simulink model "model"  (R2016a)
(part 2 of 2)

  _CN_68186251_220000_CN_281815404_220000 : powerlib/Elements/Distributed Parameters Line  Phases=3  Frequency=50  Resistance=[0.01273 0.3864]  Inductance="[0.9337e-3  4.1264e-3]"  Capacitance=[12.74e-9 7.751e-9]  Length=9.6858  x1=[8.73114913702011e-11 380000 380000;314.159265358979 314.159265358979 314.159265358979;-0.177670123217348 0.415246442777429 -1.15554988401747]  x2=[1.26090477118469e-09 381852.398472139 381852.398472139;314.159265358979 314.159265358979 314.159265358979;-1.41941675517191 0.415007521738739 -1.15578880505616]  x3=[1.07663708898761e-11 1405.24743813465 1405.24743813466;314.159265358979 314.159265358979 314.159265358979;-2.70558821102223 0.316110507002444 -1.25468581979246]  x4=[8.62234243168895e-12 1405.96374414071 1405.9637441407;314.159265358979 314.159265358979 314.159265358979;0.245769282942371 0.405640215255436 -1.16515611153945]  x5=0.000565541566995742  V1=ones(3,3)  V2=ones(3,3)  I1=ones(3,3)  I2=ones(3,3)  nHarmo=1  Measurements=None
  _CN_68186251_220000_CN_376534298_220000 : powerlib/Elements/Distributed Parameters Line  Phases=3  Frequency=50  Resistance=[0.01273 0.3864]  Inductance="[0.9337e-3  4.1264e-3]"  Capacitance=[12.74e-9 7.751e-9]  Length=7.5155  x1=[8.73114913702011e-11 380000 380000;314.159265358979 314.159265358979 314.159265358979;-0.177670123217348 0.415246442777429 -1.15554988401747]  x2=[1.26090477118469e-09 381852.398472139 381852.398472139;314.159265358979 314.159265358979 314.159265358979;-1.41941675517191 0.415007521738739 -1.15578880505616]  x3=[1.07663708898761e-11 1405.24743813465 1405.24743813466;314.159265358979 314.159265358979 314.159265358979;-2.70558821102223 0.316110507002444 -1.25468581979246]  x4=[8.62234243168895e-12 1405.96374414071 1405.9637441407;314.159265358979 314.159265358979 314.159265358979;0.245769282942371 0.405640215255436 -1.16515611153945]  x5=0.000565541566995742  V1=ones(3,3)  V2=ones(3,3)  I1=ones(3,3)  I2=ones(3,3)  nHarmo=1  Measurements=None
  _CN_71500123_220000_CN_210568055_220000 : powerlib/Elements/Distributed Parameters Line  Phases=3  Frequency=50  Resistance=[0.01273 0.3864]  Inductance="[0.9337e-3  4.1264e-3]"  Capacitance=[12.74e-9 7.751e-9]  Length=40.5732  x1=[8.73114913702011e-11 380000 380000;314.159265358979 314.159265358979 314.159265358979;-0.177670123217348 0.415246442777429 -1.15554988401747]  x2=[1.26090477118469e-09 381852.398472139 381852.398472139;314.159265358979 314.159265358979 314.159265358979;-1.41941675517191 0.415007521738739 -1.15578880505616]  x3=[1.07663708898761e-11 1405.24743813465 1405.24743813466;314.159265358979 314.159265358979 314.159265358979;-2.70558821102223 0.316110507002444 -1.25468581979246]  x4=[8.62234243168895e-12 1405.96374414071 1405.9637441407;314.159265358979 314.159265358979 314.159265358979;0.245769282942371 0.405640215255436 -1.16515611153945]  x5=0.000565541566995742  V1=ones(3,3)  V2=ones(3,3)  I1=ones(3,3)  I2=ones(3,3)  nHarmo=1  Measurements=None
  _CN_71500123_220000_CN_211907009_220000 : powerlib/Elements/Distributed Parameters Line  Phases=3  Frequency=50  Resistance=[0.01273 0.3864]  Inductance="[0.9337e-3  4.1264e-3]"  Capacitance=[12.74e-9 7.751e-9]  Length=44.7884  x1=[8.73114913702011e-11 380000 380000;314.159265358979 314.159265358979 314.159265358979;-0.177670123217348 0.415246442777429 -1.15554988401747]  x2=[1.26090477118469e-09 381852.398472139 381852.398472139;314.159265358979 314.159265358979 314.159265358979;-1.41941675517191 0.415007521738739 -1.15578880505616]  x3=[1.07663708898761e-11 1405.24743813465 1405.24743813466;314.159265358979 314.159265358979 314.159265358979;-2.70558821102223 0.316110507002444 -1.25468581979246]  x4=[8.62234243168895e-12 1405.96374414071 1405.9637441407;314.159265358979 314.159265358979 314.159265358979;0.245769282942371 0.405640215255436 -1.16515611153945]  x5=0.000565541566995742  V1=ones(3,3)  V2=ones(3,3)  I1=ones(3,3)  I2=ones(3,3)  nHarmo=1  Measurements=None
  _CN_71500123_220000_CN_36348118_220000 : powerlib/Elements/Distributed Parameters Line  Phases=3  Frequency=50  Resistance=[0.01273 0.3864]  Inductance="[0.9337e-3  4.1264e-3]"  Capacitance=[12.74e-9 7.751e-9]  Length=9.2289  x1=[8.73114913702011e-11 380000 380000;314.159265358979 314.159265358979 314.159265358979;-0.177670123217348 0.415246442777429 -1.15554988401747]  x2=[1.26090477118469e-09 381852.398472139 381852.398472139;314.159265358979 314.159265358979 314.159265358979;-1.41941675517191 0.415007521738739 -1.15578880505616]  x3=[1.07663708898761e-11 1405.24743813465 1405.24743813466;314.159265358979 314.159265358979 314.159265358979;-2.70558821102223 0.316110507002444 -1.25468581979246]  x4=[8.62234243168895e-12 1405.96374414071 1405.9637441407;314.159265358979 314.159265358979 314.159265358979;0.245769282942371 0.405640215255436 -1.16515611153945]  x5=0.000565541566995742  V1=ones(3,3)  V2=ones(3,3)  I1=ones(3,3)  I2=ones(3,3)  nHarmo=1  Measurements=None
  _CN_71500123_220000_CN_365556107_220000 : powerlib/Elements/Distributed Parameters Line  Phases=3  Frequency=50  Resistance=[0.01273 0.3864]  Inductance="[0.9337e-3  4.1264e-3]"  Capacitance=[12.74e-9 7.751e-9]  Length=24.4165  x1=[8.73114913702011e-11 380000 380000;314.159265358979 314.159265358979 314.159265358979;-0.177670123217348 0.415246442777429 -1.15554988401747]  x2=[1.26090477118469e-09 381852.398472139 381852.398472139;314.159265358979 314.159265358979 314.159265358979;-1.41941675517191 0.415007521738739 -1.15578880505616]  x3=[1.07663708898761e-11 1405.24743813465 1405.24743813466;314.159265358979 314.159265358979 314.159265358979;-2.70558821102223 0.316110507002444 -1.25468581979246]  x4=[8.62234243168895e-12 1405.96374414071 1405.9637441407;314.159265358979 314.159265358979 314.159265358979;0.245769282942371 0.405640215255436 -1.16515611153945]  x5=0.000565541566995742  V1=ones(3,3)  V2=ones(3,3)  I1=ones(3,3)  I2=ones(3,3)  nHarmo=1  Measurements=None
  _CN_71500123_380000_CN156092814 : powerlib/Elements/Distributed Parameters Line  Phases=3  Frequency=50  Resistance=[0.01273 0.3864]  Inductance="[0.9337e-3  4.1264e-3]"  Capacitance=[12.74e-9 7.751e-9]  Length=26.701  x1=[8.73114913702011e-11 380000 380000;314.159265358979 314.159265358979 314.159265358979;-0.177670123217348 0.415246442777429 -1.15554988401747]  x2=[1.26090477118469e-09 381852.398472139 381852.398472139;314.159265358979 314.159265358979 314.159265358979;-1.41941675517191 0.415007521738739 -1.15578880505616]  x3=[1.07663708898761e-11 1405.24743813465 1405.24743813466;314.159265358979 314.159265358979 314.159265358979;-2.70558821102223 0.316110507002444 -1.25468581979246]  x4=[8.62234243168895e-12 1405.96374414071 1405.9637441407;314.159265358979 314.159265358979 314.159265358979;0.245769282942371 0.405640215255436 -1.16515611153945]  x5=0.000565541566995742  V1=ones(3,3)  V2=ones(3,3)  I1=ones(3,3)  I2=ones(3,3)  nHarmo=1  Measurements=None
  _CN_80266169_220000_CN_163881972_220000 : powerlib/Elements/Distributed Parameters Line  Phases=3  Frequency=50  Resistance=[0.01273 0.3864]  Inductance="[0.9337e-3  4.1264e-3]"  Capacitance=[12.74e-9 7.751e-9]  Length=17.0488  x1=[8.73114913702011e-11 380000 380000;314.159265358979 314.159265358979 314.159265358979;-0.177670123217348 0.415246442777429 -1.15554988401747]  x2=[1.26090477118469e-09 381852.398472139 381852.398472139;314.159265358979 314.159265358979 314.159265358979;-1.41941675517191 0.415007521738739 -1.15578880505616]  x3=[1.07663708898761e-11 1405.24743813465 1405.24743813466;314.159265358979 314.159265358979 314.159265358979;-2.70558821102223 0.316110507002444 -1.25468581979246]  x4=[8.62234243168895e-12 1405.96374414071 1405.9637441407;314.159265358979 314.159265358979 314.159265358979;0.245769282942371 0.405640215255436 -1.16515611153945]  x5=0.000565541566995742  V1=ones(3,3)  V2=ones(3,3)  I1=ones(3,3)  I2=ones(3,3)  nHarmo=1  Measurements=None
  _CN_80266169_220000_CN_194258388_220000 : powerlib/Elements/Distributed Parameters Line  Phases=3  Frequency=50  Resistance=[0.01273 0.3864]  Inductance="[0.9337e-3  4.1264e-3]"  Capacitance=[12.74e-9 7.751e-9]  Length=66.2326  x1=[8.73114913702011e-11 380000 380000;314.159265358979 314.159265358979 314.159265358979;-0.177670123217348 0.415246442777429 -1.15554988401747]  x2=[1.26090477118469e-09 381852.398472139 381852.398472139;314.159265358979 314.159265358979 314.159265358979;-1.41941675517191 0.415007521738739 -1.15578880505616]  x3=[1.07663708898761e-11 1405.24743813465 1405.24743813466;314.159265358979 314.159265358979 314.159265358979;-2.70558821102223 0.316110507002444 -1.25468581979246]  x4=[8.62234243168895e-12 1405.96374414071 1405.9637441407;314.159265358979 314.159265358979 314.159265358979;0.245769282942371 0.405640215255436 -1.16515611153945]  x5=0.000565541566995742  V1=ones(3,3)  V2=ones(3,3)  I1=ones(3,3)  I2=ones(3,3)  nHarmo=1  Measurements=None
  _CN_80266169_220000_CN_34238394_220000 : powerlib/Elements/Distributed Parameters Line  Phases=3  Frequency=50  Resistance=[0.01273 0.3864]  Inductance="[0.9337e-3  4.1264e-3]"  Capacitance=[12.74e-9 7.751e-9]  Length=1.2448  x1=[8.73114913702011e-11 380000 380000;314.159265358979 314.159265358979 314.159265358979;-0.177670123217348 0.415246442777429 -1.15554988401747]  x2=[1.26090477118469e-09 381852.398472139 381852.398472139;314.159265358979 314.159265358979 314.159265358979;-1.41941675517191 0.415007521738739 -1.15578880505616]  x3=[1.07663708898761e-11 1405.24743813465 1405.24743813466;314.159265358979 314.159265358979 314.159265358979;-2.70558821102223 0.316110507002444 -1.25468581979246]  x4=[8.62234243168895e-12 1405.96374414071 1405.9637441407;314.159265358979 314.159265358979 314.159265358979;0.245769282942371 0.405640215255436 -1.16515611153945]  x5=0.000565541566995742  V1=ones(3,3)  V2=ones(3,3)  I1=ones(3,3)  I2=ones(3,3)  nHarmo=1  Measurements=None
  _CN_89405664_220000_CN_190819048_220000 : powerlib/Elements/Distributed Parameters Line  Phases=3  Frequency=50  Resistance=[0.01273 0.3864]  Inductance="[0.9337e-3  4.1264e-3]"  Capacitance=[12.74e-9 7.751e-9]  Length=27.3541  x1=[8.73114913702011e-11 380000 380000;314.159265358979 314.159265358979 314.159265358979;-0.177670123217348 0.415246442777429 -1.15554988401747]  x2=[1.26090477118469e-09 381852.398472139 381852.398472139;314.159265358979 314.159265358979 314.159265358979;-1.41941675517191 0.415007521738739 -1.15578880505616]  x3=[1.07663708898761e-11 1405.24743813465 1405.24743813466;314.159265358979 314.159265358979 314.159265358979;-2.70558821102223 0.316110507002444 -1.25468581979246]  x4=[8.62234243168895e-12 1405.96374414071 1405.9637441407;314.159265358979 314.159265358979 314.159265358979;0.245769282942371 0.405640215255436 -1.16515611153945]  x5=0.000565541566995742  V1=ones(3,3)  V2=ones(3,3)  I1=ones(3,3)  I2=ones(3,3)  nHarmo=1  Measurements=None
  _CN_89977424_380000_CN_195751829_380000 : powerlib/Elements/Distributed Parameters Line  Phases=3  Frequency=50  Resistance=[0.01273 0.3864]  Inductance="[0.9337e-3  4.1264e-3]"  Capacitance=[12.74e-9 7.751e-9]  Length=3.0406  x1=[8.73114913702011e-11 380000 380000;314.159265358979 314.159265358979 314.159265358979;-0.177670123217348 0.415246442777429 -1.15554988401747]  x2=[1.26090477118469e-09 381852.398472139 381852.398472139;314.159265358979 314.159265358979 314.159265358979;-1.41941675517191 0.415007521738739 -1.15578880505616]  x3=[1.07663708898761e-11 1405.24743813465 1405.24743813466;314.159265358979 314.159265358979 314.159265358979;-2.70558821102223 0.316110507002444 -1.25468581979246]  x4=[8.62234243168895e-12 1405.96374414071 1405.9637441407;314.159265358979 314.159265358979 314.159265358979;0.245769282942371 0.405640215255436 -1.16515611153945]  x5=0.000565541566995742  V1=ones(3,3)  V2=ones(3,3)  I1=ones(3,3)  I2=ones(3,3)  nHarmo=1  Measurements=None
  _CN_89977424_380000_CN_31308888_380000 : powerlib/Elements/Distributed Parameters Line  Phases=3  Frequency=50  Resistance=[0.01273 0.3864]  Inductance="[0.9337e-3  4.1264e-3]"  Capacitance=[12.74e-9 7.751e-9]  Length=10.6473  x1=[8.73114913702011e-11 380000 380000;314.159265358979 314.159265358979 314.159265358979;-0.177670123217348 0.415246442777429 -1.15554988401747]  x2=[1.26090477118469e-09 381852.398472139 381852.398472139;314.159265358979 314.159265358979 314.159265358979;-1.41941675517191 0.415007521738739 -1.15578880505616]  x3=[1.07663708898761e-11 1405.24743813465 1405.24743813466;314.159265358979 314.159265358979 314.159265358979;-2.70558821102223 0.316110507002444 -1.25468581979246]  x4=[8.62234243168895e-12 1405.96374414071 1405.9637441407;314.159265358979 314.159265358979 314.159265358979;0.245769282942371 0.405640215255436 -1.16515611153945]  x5=0.000565541566995742  V1=ones(3,3)  V2=ones(3,3)  I1=ones(3,3)  I2=ones(3,3)  nHarmo=1  Measurements=None
  _CN_97941869_380000_CN_35002638_380000 : powerlib/Elements/Distributed Parameters Line  Phases=3  Frequency=50  Resistance=[0.01273 0.3864]  Inductance="[0.9337e-3  4.1264e-3]"  Capacitance=[12.74e-9 7.751e-9]  Length=18.8024  x1=[8.73114913702011e-11 380000 380000;314.159265358979 314.159265358979 314.159265358979;-0.177670123217348 0.415246442777429 -1.15554988401747]  x2=[1.26090477118469e-09 381852.398472139 381852.398472139;314.159265358979 314.159265358979 314.159265358979;-1.41941675517191 0.415007521738739 -1.15578880505616]  x3=[1.07663708898761e-11 1405.24743813465 1405.24743813466;314.159265358979 314.159265358979 314.159265358979;-2.70558821102223 0.316110507002444 -1.25468581979246]  x4=[8.62234243168895e-12 1405.96374414071 1405.9637441407;314.159265358979 314.159265358979 314.159265358979;0.245769282942371 0.405640215255436 -1.16515611153945]  x5=0.000565541566995742  V1=ones(3,3)  V2=ones(3,3)  I1=ones(3,3)  I2=ones(3,3)  nHarmo=1  Measurements=None
  _CN_98648381_220000_CN_27107779_220000 : powerlib/Elements/Distributed Parameters Line  Phases=3  Frequency=50  Resistance=[0.01273 0.3864]  Inductance="[0.9337e-3  4.1264e-3]"  Capacitance=[12.74e-9 7.751e-9]  Length=59.2829  x1=[8.73114913702011e-11 380000 380000;314.159265358979 314.159265358979 314.159265358979;-0.177670123217348 0.415246442777429 -1.15554988401747]  x2=[1.26090477118469e-09 381852.398472139 381852.398472139;314.159265358979 314.159265358979 314.159265358979;-1.41941675517191 0.415007521738739 -1.15578880505616]  x3=[1.07663708898761e-11 1405.24743813465 1405.24743813466;314.159265358979 314.159265358979 314.159265358979;-2.70558821102223 0.316110507002444 -1.25468581979246]  x4=[8.62234243168895e-12 1405.96374414071 1405.9637441407;314.159265358979 314.159265358979 314.159265358979;0.245769282942371 0.405640215255436 -1.16515611153945]  x5=0.000565541566995742  V1=ones(3,3)  V2=ones(3,3)  I1=ones(3,3)  I2=ones(3,3)  nHarmo=1  Measurements=None
  _CN_98648381_220000_CN_50319857_220000 : powerlib/Elements/Distributed Parameters Line  Phases=3  Frequency=50  Resistance=[0.01273 0.3864]  Inductance="[0.9337e-3  4.1264e-3]"  Capacitance=[12.74e-9 7.751e-9]  Length=22.8534  x1=[8.73114913702011e-11 380000 380000;314.159265358979 314.159265358979 314.159265358979;-0.177670123217348 0.415246442777429 -1.15554988401747]  x2=[1.26090477118469e-09 381852.398472139 381852.398472139;314.159265358979 314.159265358979 314.159265358979;-1.41941675517191 0.415007521738739 -1.15578880505616]  x3=[1.07663708898761e-11 1405.24743813465 1405.24743813466;314.159265358979 314.159265358979 314.159265358979;-2.70558821102223 0.316110507002444 -1.25468581979246]  x4=[8.62234243168895e-12 1405.96374414071 1405.9637441407;314.159265358979 314.159265358979 314.159265358979;0.245769282942371 0.405640215255436 -1.16515611153945]  x5=0.000565541566995742  V1=ones(3,3)  V2=ones(3,3)  I1=ones(3,3)  I2=ones(3,3)  nHarmo=1  Measurements=None
  _CN_98648381_380000_CN_147714395_380000 : powerlib/Elements/Distributed Parameters Line  Phases=3  Frequency=50  Resistance=[0.01273 0.3864]  Inductance="[0.9337e-3  4.1264e-3]"  Capacitance=[12.74e-9 7.751e-9]  Length=59.2296  x1=[8.73114913702011e-11 380000 380000;314.159265358979 314.159265358979 314.159265358979;-0.177670123217348 0.415246442777429 -1.15554988401747]  x2=[1.26090477118469e-09 381852.398472139 381852.398472139;314.159265358979 314.159265358979 314.159265358979;-1.41941675517191 0.415007521738739 -1.15578880505616]  x3=[1.07663708898761e-11 1405.24743813465 1405.24743813466;314.159265358979 314.159265358979 314.159265358979;-2.70558821102223 0.316110507002444 -1.25468581979246]  x4=[8.62234243168895e-12 1405.96374414071 1405.9637441407;314.159265358979 314.159265358979 314.159265358979;0.245769282942371 0.405640215255436 -1.16515611153945]  x5=0.000565541566995742  V1=ones(3,3)  V2=ones(3,3)  I1=ones(3,3)  I2=ones(3,3)  nHarmo=1  Measurements=None
  _CN_98648381_380000_CN_50319857_380000 : powerlib/Elements/Distributed Parameters Line  Phases=3  Frequency=50  Resistance=[0.01273 0.3864]  Inductance="[0.9337e-3  4.1264e-3]"  Capacitance=[12.74e-9 7.751e-9]  Length=22.6956  x1=[8.73114913702011e-11 380000 380000;314.159265358979 314.159265358979 314.159265358979;-0.177670123217348 0.415246442777429 -1.15554988401747]  x2=[1.26090477118469e-09 381852.398472139 381852.398472139;314.159265358979 314.159265358979 314.159265358979;-1.41941675517191 0.415007521738739 -1.15578880505616]  x3=[1.07663708898761e-11 1405.24743813465 1405.24743813466;314.159265358979 314.159265358979 314.159265358979;-2.70558821102223 0.316110507002444 -1.25468581979246]  x4=[8.62234243168895e-12 1405.96374414071 1405.9637441407;314.159265358979 314.159265358979 314.159265358979;0.245769282942371 0.405640215255436 -1.16515611153945]  x5=0.000565541566995742  V1=ones(3,3)  V2=ones(3,3)  I1=ones(3,3)  I2=ones(3,3)  nHarmo=1  Measurements=None
  bus1 : powerlib/Measurements/Load Flow Bus  LConnTagsString=a  Phases=single  Connectors=on one side  ID=bus1  Vbase=220000  Vref=1  Vangle=0  VLF=1  VLFb=1  VLFc=1  angleLF=0  angleLFb=0  angleLFc=0
      settings: AttributesFormatString=|
      | %<ID>
      | %<Vbase>V
      | %<VLF>pu
      | %<angleLF>deg.
      | %<Name>
  bus10 : powerlib/Measurements/Load Flow Bus  LConnTagsString=a  Phases=single  Connectors=on one side  ID=bus10  Vbase=220000  Vref=1  Vangle=0  VLF=1  VLFb=1  VLFc=1  angleLF=0  angleLFb=0  angleLFc=0
      settings: AttributesFormatString=|
      | %<ID>
      | %<Vbase>V
      | %<VLF>pu
      | %<angleLF>deg.
      | %<Name>
  bus100 : powerlib/Measurements/Load Flow Bus  LConnTagsString=a  Phases=single  Connectors=on one side  ID=bus100  Vbase=220000  Vref=1  Vangle=0  VLF=1  VLFb=1  VLFc=1  angleLF=0  angleLFb=0  angleLFc=0
      settings: AttributesFormatString=|
      | %<ID>
      | %<Vbase>V
      | %<VLF>pu
      | %<angleLF>deg.
      | %<Name>
  bus101 : powerlib/Measurements/Load Flow Bus  LConnTagsString=a  Phases=single  Connectors=on one side  ID=bus101  Vbase=220000  Vref=1  Vangle=0  VLF=1  VLFb=1  VLFc=1  angleLF=0  angleLFb=0  angleLFc=0
      settings: AttributesFormatString=|
      | %<ID>
      | %<Vbase>V
      | %<VLF>pu
      | %<angleLF>deg.
      | %<Name>
  bus102 : powerlib/Measurements/Load Flow Bus  LConnTagsString=a  Phases=single  Connectors=on one side  ID=bus102  Vbase=220000  Vref=1  Vangle=0  VLF=1  VLFb=1  VLFc=1  angleLF=0  angleLFb=0  angleLFc=0
      settings: AttributesFormatString=|
      | %<ID>
      | %<Vbase>V
      | %<VLF>pu
      | %<angleLF>deg.
      | %<Name>
  bus103 : powerlib/Measurements/Load Flow Bus  LConnTagsString=a  Phases=single  Connectors=on one side  ID=bus103  Vbase=220000  Vref=1  Vangle=0  VLF=1  VLFb=1  VLFc=1  angleLF=0  angleLFb=0  angleLFc=0
      settings: AttributesFormatString=|
      | %<ID>
      | %<Vbase>V
      | %<VLF>pu
      | %<angleLF>deg.
      | %<Name>
  bus104 : powerlib/Measurements/Load Flow Bus  LConnTagsString=a  Phases=single  Connectors=on one side  ID=bus104  Vbase=220000  Vref=1  Vangle=0  VLF=1  VLFb=1  VLFc=1  angleLF=0  angleLFb=0  angleLFc=0
      settings: AttributesFormatString=|
      | %<ID>
      | %<Vbase>V
      | %<VLF>pu
      | %<angleLF>deg.
      | %<Name>
  bus105 : powerlib/Measurements/Load Flow Bus  LConnTagsString=a  Phases=single  Connectors=on one side  ID=bus105  Vbase=220000  Vref=1  Vangle=0  VLF=1  VLFb=1  VLFc=1  angleLF=0  angleLFb=0  angleLFc=0
      settings: AttributesFormatString=|
      | %<ID>
      | %<Vbase>V
      | %<VLF>pu
      | %<angleLF>deg.
      | %<Name>
  bus106 : powerlib/Measurements/Load Flow Bus  LConnTagsString=a  Phases=single  Connectors=on one side  ID=bus106  Vbase=380000  Vref=1  Vangle=0  VLF=1  VLFb=1  VLFc=1  angleLF=0  angleLFb=0  angleLFc=0
      settings: AttributesFormatString=|
      | %<ID>
      | %<Vbase>V
      | %<VLF>pu
      | %<angleLF>deg.
      | %<Name>
  bus107 : powerlib/Measurements/Load Flow Bus  LConnTagsString=a  Phases=single  Connectors=on one side  ID=bus107  Vbase=220000  Vref=1  Vangle=0  VLF=1  VLFb=1  VLFc=1  angleLF=0  angleLFb=0  angleLFc=0
      settings: AttributesFormatString=|
      | %<ID>
      | %<Vbase>V
      | %<VLF>pu
      | %<angleLF>deg.
      | %<Name>
  bus108 : powerlib/Measurements/Load Flow Bus  LConnTagsString=a  Phases=single  Connectors=on one side  ID=bus108  Vbase=220000  Vref=1  Vangle=0  VLF=1  VLFb=1  VLFc=1  angleLF=0  angleLFb=0  angleLFc=0
      settings: AttributesFormatString=|
      | %<ID>
      | %<Vbase>V
      | %<VLF>pu
      | %<angleLF>deg.
      | %<Name>
  bus109 : powerlib/Measurements/Load Flow Bus  LConnTagsString=a  Phases=single  Connectors=on one side  ID=bus109  Vbase=220000  Vref=1  Vangle=0  VLF=1  VLFb=1  VLFc=1  angleLF=0  angleLFb=0  angleLFc=0
      settings: AttributesFormatString=|
      | %<ID>
      | %<Vbase>V
      | %<VLF>pu
      | %<angleLF>deg.
      | %<Name>
  bus11 : powerlib/Measurements/Load Flow Bus  LConnTagsString=a  Phases=single  Connectors=on one side  ID=bus11  Vbase=220000  Vref=1  Vangle=0  VLF=1  VLFb=1  VLFc=1  angleLF=0  angleLFb=0  angleLFc=0
      settings: AttributesFormatString=|
      | %<ID>
      | %<Vbase>V
      | %<VLF>pu
      | %<angleLF>deg.
      | %<Name>
  bus110 : powerlib/Measurements/Load Flow Bus  LConnTagsString=a  Phases=single  Connectors=on one side  ID=bus110  Vbase=220000  Vref=1  Vangle=0  VLF=1  VLFb=1  VLFc=1  angleLF=0  angleLFb=0  angleLFc=0
      settings: AttributesFormatString=|
      | %<ID>
      | %<Vbase>V
      | %<VLF>pu
      | %<angleLF>deg.
      | %<Name>
  bus111 : powerlib/Measurements/Load Flow Bus  LConnTagsString=a  Phases=single  Connectors=on one side  ID=bus111  Vbase=380000  Vref=1  Vangle=0  VLF=1  VLFb=1  VLFc=1  angleLF=0  angleLFb=0  angleLFc=0
      settings: AttributesFormatString=|
      | %<ID>
      | %<Vbase>V
      | %<VLF>pu
      | %<angleLF>deg.
      | %<Name>
  bus112 : powerlib/Measurements/Load Flow Bus  LConnTagsString=a  Phases=single  Connectors=on one side  ID=bus112  Vbase=380000  Vref=1  Vangle=0  VLF=1  VLFb=1  VLFc=1  angleLF=0  angleLFb=0  angleLFc=0
      settings: AttributesFormatString=|
      | %<ID>
      | %<Vbase>V
      | %<VLF>pu
      | %<angleLF>deg.
      | %<Name>
  bus113 : powerlib/Measurements/Load Flow Bus  LConnTagsString=a  Phases=single  Connectors=on one side  ID=bus113  Vbase=220000  Vref=1  Vangle=0  VLF=1  VLFb=1  VLFc=1  angleLF=0  angleLFb=0  angleLFc=0
      settings: AttributesFormatString=|
      | %<ID>
      | %<Vbase>V
      | %<VLF>pu
      | %<angleLF>deg.
      | %<Name>
  bus114 : powerlib/Measurements/Load Flow Bus  LConnTagsString=a  Phases=single  Connectors=on one side  ID=bus114  Vbase=220000  Vref=1  Vangle=0  VLF=1  VLFb=1  VLFc=1  angleLF=0  angleLFb=0  angleLFc=0
      settings: AttributesFormatString=|
      | %<ID>
      | %<Vbase>V
      | %<VLF>pu
      | %<angleLF>deg.
      | %<Name>
  bus115 : powerlib/Measurements/Load Flow Bus  LConnTagsString=a  Phases=single  Connectors=on one side  ID=bus115  Vbase=220000  Vref=1  Vangle=0  VLF=1  VLFb=1  VLFc=1  angleLF=0  angleLFb=0  angleLFc=0
      settings: AttributesFormatString=|
      | %<ID>
      | %<Vbase>V
      | %<VLF>pu
      | %<angleLF>deg.
      | %<Name>
  bus116 : powerlib/Measurements/Load Flow Bus  LConnTagsString=a  Phases=single  Connectors=on one side  ID=bus116  Vbase=220000  Vref=1  Vangle=0  VLF=1  VLFb=1  VLFc=1  angleLF=0  angleLFb=0  angleLFc=0
      settings: AttributesFormatString=|
      | %<ID>
      | %<Vbase>V
      | %<VLF>pu
      | %<angleLF>deg.
      | %<Name>
  bus117 : powerlib/Measurements/Load Flow Bus  LConnTagsString=a  Phases=single  Connectors=on one side  ID=bus117  Vbase=220000  Vref=1  Vangle=0  VLF=1  VLFb=1  VLFc=1  angleLF=0  angleLFb=0  angleLFc=0
      settings: AttributesFormatString=|
      | %<ID>
      | %<Vbase>V
      | %<VLF>pu
      | %<angleLF>deg.
      | %<Name>
  bus118 : powerlib/Measurements/Load Flow Bus  LConnTagsString=a  Phases=single  Connectors=on one side  ID=bus118  Vbase=220000  Vref=1  Vangle=0  VLF=1  VLFb=1  VLFc=1  angleLF=0  angleLFb=0  angleLFc=0
      settings: AttributesFormatString=|
      | %<ID>
      | %<Vbase>V
      | %<VLF>pu
      | %<angleLF>deg.
      | %<Name>
  bus119 : powerlib/Measurements/Load Flow Bus  LConnTagsString=a  Phases=single  Connectors=on one side  ID=bus119  Vbase=220000  Vref=1  Vangle=0  VLF=1  VLFb=1  VLFc=1  angleLF=0  angleLFb=0  angleLFc=0
      settings: AttributesFormatString=|
      | %<ID>
      | %<Vbase>V
      | %<VLF>pu
      | %<angleLF>deg.
      | %<Name>
  bus12 : powerlib/Measurements/Load Flow Bus  LConnTagsString=a  Phases=single  Connectors=on one side  ID=bus12  Vbase=220000  Vref=1  Vangle=0  VLF=1  VLFb=1  VLFc=1  angleLF=0  angleLFb=0  angleLFc=0
      settings: AttributesFormatString=|
      | %<ID>
      | %<Vbase>V
      | %<VLF>pu
      | %<angleLF>deg.
      | %<Name>
  bus120 : powerlib/Measurements/Load Flow Bus  LConnTagsString=a  Phases=single  Connectors=on one side  ID=bus120  Vbase=220000  Vref=1  Vangle=0  VLF=1  VLFb=1  VLFc=1  angleLF=0  angleLFb=0  angleLFc=0
      settings: AttributesFormatString=|
      | %<ID>
      | %<Vbase>V
      | %<VLF>pu
      | %<angleLF>deg.
      | %<Name>
  bus121 : powerlib/Measurements/Load Flow Bus  LConnTagsString=a  Phases=single  Connectors=on one side  ID=bus121  Vbase=220000  Vref=1  Vangle=0  VLF=1  VLFb=1  VLFc=1  angleLF=0  angleLFb=0  angleLFc=0
      settings: AttributesFormatString=|
      | %<ID>
      | %<Vbase>V
      | %<VLF>pu
      | %<angleLF>deg.
      | %<Name>
  bus122 : powerlib/Measurements/Load Flow Bus  LConnTagsString=a  Phases=single  Connectors=on one side  ID=bus122  Vbase=220000  Vref=1  Vangle=0  VLF=1  VLFb=1  VLFc=1  angleLF=0  angleLFb=0  angleLFc=0
      settings: AttributesFormatString=|
      | %<ID>
      | %<Vbase>V
      | %<VLF>pu
      | %<angleLF>deg.
      | %<Name>
  bus123 : powerlib/Measurements/Load Flow Bus  LConnTagsString=a  Phases=single  Connectors=on one side  ID=bus123  Vbase=220000  Vref=1  Vangle=0  VLF=1  VLFb=1  VLFc=1  angleLF=0  angleLFb=0  angleLFc=0
      settings: AttributesFormatString=|
      | %<ID>
      | %<Vbase>V
      | %<VLF>pu
      | %<angleLF>deg.
      | %<Name>
  bus124 : powerlib/Measurements/Load Flow Bus  LConnTagsString=a  Phases=single  Connectors=on one side  ID=bus124  Vbase=220000  Vref=1  Vangle=0  VLF=1  VLFb=1  VLFc=1  angleLF=0  angleLFb=0  angleLFc=0
      settings: AttributesFormatString=|
      | %<ID>
      | %<Vbase>V
      | %<VLF>pu
      | %<angleLF>deg.
      | %<Name>
  bus125 : powerlib/Measurements/Load Flow Bus  LConnTagsString=a  Phases=single  Connectors=on one side  ID=bus125  Vbase=220000  Vref=1  Vangle=0  VLF=1  VLFb=1  VLFc=1  angleLF=0  angleLFb=0  angleLFc=0
      settings: AttributesFormatString=|
      | %<ID>
      | %<Vbase>V
      | %<VLF>pu
      | %<angleLF>deg.
      | %<Name>
  bus126 : powerlib/Measurements/Load Flow Bus  LConnTagsString=a  Phases=single  Connectors=on one side  ID=bus126  Vbase=220000  Vref=1  Vangle=0  VLF=1  VLFb=1  VLFc=1  angleLF=0  angleLFb=0  angleLFc=0
      settings: AttributesFormatString=|
      | %<ID>
      | %<Vbase>V
      | %<VLF>pu
      | %<angleLF>deg.
      | %<Name>
  bus127 : powerlib/Measurements/Load Flow Bus  LConnTagsString=a  Phases=single  Connectors=on one side  ID=bus127  Vbase=220000  Vref=1  Vangle=0  VLF=1  VLFb=1  VLFc=1  angleLF=0  angleLFb=0  angleLFc=0
      settings: AttributesFormatString=|
      | %<ID>
      | %<Vbase>V
      | %<VLF>pu
      | %<angleLF>deg.
      | %<Name>
  bus128 : powerlib/Measurements/Load Flow Bus  LConnTagsString=a  Phases=single  Connectors=on one side  ID=bus128  Vbase=220000  Vref=1  Vangle=0  VLF=1  VLFb=1  VLFc=1  angleLF=0  angleLFb=0  angleLFc=0
      settings: AttributesFormatString=|
      | %<ID>
      | %<Vbase>V
      | %<VLF>pu
      | %<angleLF>deg.
      | %<Name>
  bus129 : powerlib/Measurements/Load Flow Bus  LConnTagsString=a  Phases=single  Connectors=on one side  ID=bus129  Vbase=220000  Vref=1  Vangle=0  VLF=1  VLFb=1  VLFc=1  angleLF=0  angleLFb=0  angleLFc=0
      settings: AttributesFormatString=|
      | %<ID>
      | %<Vbase>V
      | %<VLF>pu
      | %<angleLF>deg.
      | %<Name>
  bus13 : powerlib/Measurements/Load Flow Bus  LConnTagsString=a  Phases=single  Connectors=on one side  ID=bus13  Vbase=220000  Vref=1  Vangle=0  VLF=1  VLFb=1  VLFc=1  angleLF=0  angleLFb=0  angleLFc=0
      settings: AttributesFormatString=|
      | %<ID>
      | %<Vbase>V
      | %<VLF>pu
      | %<angleLF>deg.
      | %<Name>
  bus130 : powerlib/Measurements/Load Flow Bus  LConnTagsString=a  Phases=single  Connectors=on one side  ID=bus130  Vbase=220000  Vref=1  Vangle=0  VLF=1  VLFb=1  VLFc=1  angleLF=0  angleLFb=0  angleLFc=0
      settings: AttributesFormatString=|
      | %<ID>
      | %<Vbase>V
      | %<VLF>pu
      | %<angleLF>deg.
      | %<Name>
  bus131 : powerlib/Measurements/Load Flow Bus  LConnTagsString=a  Phases=single  Connectors=on one side  ID=bus131  Vbase=220000  Vref=1  Vangle=0  VLF=1  VLFb=1  VLFc=1  angleLF=0  angleLFb=0  angleLFc=0
      settings: AttributesFormatString=|
      | %<ID>
      | %<Vbase>V
      | %<VLF>pu
      | %<angleLF>deg.
      | %<Name>
  bus132 : powerlib/Measurements/Load Flow Bus  LConnTagsString=a  Phases=single  Connectors=on one side  ID=bus132  Vbase=220000  Vref=1  Vangle=0  VLF=1  VLFb=1  VLFc=1  angleLF=0  angleLFb=0  angleLFc=0
      settings: AttributesFormatString=|
      | %<ID>
      | %<Vbase>V
      | %<VLF>pu
      | %<angleLF>deg.
      | %<Name>
  bus133 : powerlib/Measurements/Load Flow Bus  LConnTagsString=a  Phases=single  Connectors=on one side  ID=bus133  Vbase=220000  Vref=1  Vangle=0  VLF=1  VLFb=1  VLFc=1  angleLF=0  angleLFb=0  angleLFc=0
      settings: AttributesFormatString=|
      | %<ID>
      | %<Vbase>V
      | %<VLF>pu
      | %<angleLF>deg.
      | %<Name>
  bus134 : powerlib/Measurements/Load Flow Bus  LConnTagsString=a  Phases=single  Connectors=on one side  ID=bus134  Vbase=380000  Vref=1  Vangle=0  VLF=1  VLFb=1  VLFc=1  angleLF=0  angleLFb=0  angleLFc=0
      settings: AttributesFormatString=|
      | %<ID>
      | %<Vbase>V
      | %<VLF>pu
      | %<angleLF>deg.
      | %<Name>
  bus135 : powerlib/Measurements/Load Flow Bus  LConnTagsString=a  Phases=single  Connectors=on one side  ID=bus135  Vbase=380000  Vref=1  Vangle=0  VLF=1  VLFb=1  VLFc=1  angleLF=0  angleLFb=0  angleLFc=0
      settings: AttributesFormatString=|
      | %<ID>
      | %<Vbase>V
      | %<VLF>pu
      | %<angleLF>deg.
      | %<Name>
  bus136 : powerlib/Measurements/Load Flow Bus  LConnTagsString=a  Phases=single  Connectors=on one side  ID=bus136  Vbase=380000  Vref=1  Vangle=0  VLF=1  VLFb=1  VLFc=1  angleLF=0  angleLFb=0  angleLFc=0
      settings: AttributesFormatString=|
      | %<ID>
      | %<Vbase>V
      | %<VLF>pu
      | %<angleLF>deg.
      | %<Name>
  bus137 : powerlib/Measurements/Load Flow Bus  LConnTagsString=a  Phases=single  Connectors=on one side  ID=bus137  Vbase=220000  Vref=1  Vangle=0  VLF=1  VLFb=1  VLFc=1  angleLF=0  angleLFb=0  angleLFc=0
      settings: AttributesFormatString=|
      | %<ID>
      | %<Vbase>V
      | %<VLF>pu
      | %<angleLF>deg.
      | %<Name>
  bus138 : powerlib/Measurements/Load Flow Bus  LConnTagsString=a  Phases=single  Connectors=on one side  ID=bus138  Vbase=220000  Vref=1  Vangle=0  VLF=1  VLFb=1  VLFc=1  angleLF=0  angleLFb=0  angleLFc=0
      settings: AttributesFormatString=|
      | %<ID>
      | %<Vbase>V
      | %<VLF>pu
      | %<angleLF>deg.
      | %<Name>
  bus139 : powerlib/Measurements/Load Flow Bus  LConnTagsString=a  Phases=single  Connectors=on one side  ID=bus139  Vbase=220000  Vref=1  Vangle=0  VLF=1  VLFb=1  VLFc=1  angleLF=0  angleLFb=0  angleLFc=0
      settings: AttributesFormatString=|
      | %<ID>
      | %<Vbase>V
      | %<VLF>pu
      | %<angleLF>deg.
      | %<Name>
  bus14 : powerlib/Measurements/Load Flow Bus  LConnTagsString=a  Phases=single  Connectors=on one side  ID=bus14  Vbase=220000  Vref=1  Vangle=0  VLF=1  VLFb=1  VLFc=1  angleLF=0  angleLFb=0  angleLFc=0
      settings: AttributesFormatString=|
      | %<ID>
      | %<Vbase>V
      | %<VLF>pu
      | %<angleLF>deg.
      | %<Name>
  bus140 : powerlib/Measurements/Load Flow Bus  LConnTagsString=a  Phases=single  Connectors=on one side  ID=bus140  Vbase=220000  Vref=1  Vangle=0  VLF=1  VLFb=1  VLFc=1  angleLF=0  angleLFb=0  angleLFc=0
      settings: AttributesFormatString=|
      | %<ID>
      | %<Vbase>V
      | %<VLF>pu
      | %<angleLF>deg.
      | %<Name>
  bus141 : powerlib/Measurements/Load Flow Bus  LConnTagsString=a  Phases=single  Connectors=on one side  ID=bus141  Vbase=220000  Vref=1  Vangle=0  VLF=1  VLFb=1  VLFc=1  angleLF=0  angleLFb=0  angleLFc=0
      settings: AttributesFormatString=|
      | %<ID>
      | %<Vbase>V
      | %<VLF>pu
      | %<angleLF>deg.
      | %<Name>
  bus142 : powerlib/Measurements/Load Flow Bus  LConnTagsString=a  Phases=single  Connectors=on one side  ID=bus142  Vbase=220000  Vref=1  Vangle=0  VLF=1  VLFb=1  VLFc=1  angleLF=0  angleLFb=0  angleLFc=0
      settings: AttributesFormatString=|
      | %<ID>
      | %<Vbase>V
      | %<VLF>pu
      | %<angleLF>deg.
      | %<Name>
  bus143 : powerlib/Measurements/Load Flow Bus  LConnTagsString=a  Phases=single  Connectors=on one side  ID=bus143  Vbase=220000  Vref=1  Vangle=0  VLF=1  VLFb=1  VLFc=1  angleLF=0  angleLFb=0  angleLFc=0
      settings: AttributesFormatString=|
      | %<ID>
      | %<Vbase>V
      | %<VLF>pu
      | %<angleLF>deg.
      | %<Name>
  bus144 : powerlib/Measurements/Load Flow Bus  LConnTagsString=a  Phases=single  Connectors=on one side  ID=bus144  Vbase=220000  Vref=1  Vangle=0  VLF=1  VLFb=1  VLFc=1  angleLF=0  angleLFb=0  angleLFc=0
      settings: AttributesFormatString=|
      | %<ID>
      | %<Vbase>V
      | %<VLF>pu
      | %<angleLF>deg.
      | %<Name>
  bus145 : powerlib/Measurements/Load Flow Bus  LConnTagsString=a  Phases=single  Connectors=on one side  ID=bus145  Vbase=220000  Vref=1  Vangle=0  VLF=1  VLFb=1  VLFc=1  angleLF=0  angleLFb=0  angleLFc=0
      settings: AttributesFormatString=|
      | %<ID>
      | %<Vbase>V
      | %<VLF>pu
      | %<angleLF>deg.
      | %<Name>
  bus146 : powerlib/Measurements/Load Flow Bus  LConnTagsString=a  Phases=single  Connectors=on one side  ID=bus146  Vbase=220000  Vref=1  Vangle=0  VLF=1  VLFb=1  VLFc=1  angleLF=0  angleLFb=0  angleLFc=0
      settings: AttributesFormatString=|
      | %<ID>
      | %<Vbase>V
      | %<VLF>pu
      | %<angleLF>deg.
      | %<Name>
  bus147 : powerlib/Measurements/Load Flow Bus  LConnTagsString=a  Phases=single  Connectors=on one side  ID=bus147  Vbase=220000  Vref=1  Vangle=0  VLF=1  VLFb=1  VLFc=1  angleLF=0  angleLFb=0  angleLFc=0
      settings: AttributesFormatString=|
      | %<ID>
      | %<Vbase>V
      | %<VLF>pu
      | %<angleLF>deg.
      | %<Name>
  bus148 : powerlib/Measurements/Load Flow Bus  LConnTagsString=a  Phases=single  Connectors=on one side  ID=bus148  Vbase=380000  Vref=1  Vangle=0  VLF=1  VLFb=1  VLFc=1  angleLF=0  angleLFb=0  angleLFc=0
      settings: AttributesFormatString=|
      | %<ID>
      | %<Vbase>V
      | %<VLF>pu
      | %<angleLF>deg.
      | %<Name>
  bus149 : powerlib/Measurements/Load Flow Bus  LConnTagsString=a  Phases=single  Connectors=on one side  ID=bus149  Vbase=220000  Vref=1  Vangle=0  VLF=1  VLFb=1  VLFc=1  angleLF=0  angleLFb=0  angleLFc=0
      settings: AttributesFormatString=|
      | %<ID>
      | %<Vbase>V
      | %<VLF>pu
      | %<angleLF>deg.
      | %<Name>
  bus15 : powerlib/Measurements/Load Flow Bus  LConnTagsString=a  Phases=single  Connectors=on one side  ID=bus15  Vbase=220000  Vref=1  Vangle=0  VLF=1  VLFb=1  VLFc=1  angleLF=0  angleLFb=0  angleLFc=0
      settings: AttributesFormatString=|
      | %<ID>
      | %<Vbase>V
      | %<VLF>pu
      | %<angleLF>deg.
      | %<Name>
  bus150 : powerlib/Measurements/Load Flow Bus  LConnTagsString=a  Phases=single  Connectors=on one side  ID=bus150  Vbase=220000  Vref=1  Vangle=0  VLF=1  VLFb=1  VLFc=1  angleLF=0  angleLFb=0  angleLFc=0
      settings: AttributesFormatString=|
      | %<ID>
      | %<Vbase>V
      | %<VLF>pu
      | %<angleLF>deg.
      | %<Name>
  bus151 : powerlib/Measurements/Load Flow Bus  LConnTagsString=a  Phases=single  Connectors=on one side  ID=bus151  Vbase=220000  Vref=1  Vangle=0  VLF=1  VLFb=1  VLFc=1  angleLF=0  angleLFb=0  angleLFc=0
      settings: AttributesFormatString=|
      | %<ID>
      | %<Vbase>V
      | %<VLF>pu
      | %<angleLF>deg.
      | %<Name>
  bus152 : powerlib/Measurements/Load Flow Bus  LConnTagsString=a  Phases=single  Connectors=on one side  ID=bus152  Vbase=220000  Vref=1  Vangle=0  VLF=1  VLFb=1  VLFc=1  angleLF=0  angleLFb=0  angleLFc=0
      settings: AttributesFormatString=|
      | %<ID>
      | %<Vbase>V
      | %<VLF>pu
      | %<angleLF>deg.
      | %<Name>
  bus153 : powerlib/Measurements/Load Flow Bus  LConnTagsString=a  Phases=single  Connectors=on one side  ID=bus153  Vbase=380000  Vref=1  Vangle=0  VLF=1  VLFb=1  VLFc=1  angleLF=0  angleLFb=0  angleLFc=0
      settings: AttributesFormatString=|
      | %<ID>
      | %<Vbase>V
      | %<VLF>pu
      | %<angleLF>deg.
      | %<Name>
  bus154 : powerlib/Measurements/Load Flow Bus  LConnTagsString=a  Phases=single  Connectors=on one side  ID=bus154  Vbase=380000  Vref=1  Vangle=0  VLF=1  VLFb=1  VLFc=1  angleLF=0  angleLFb=0  angleLFc=0
      settings: AttributesFormatString=|
      | %<ID>
      | %<Vbase>V
      | %<VLF>pu
      | %<angleLF>deg.
      | %<Name>
  bus155 : powerlib/Measurements/Load Flow Bus  LConnTagsString=a  Phases=single  Connectors=on one side  ID=bus155  Vbase=380000  Vref=1  Vangle=0  VLF=1  VLFb=1  VLFc=1  angleLF=0  angleLFb=0  angleLFc=0
      settings: AttributesFormatString=|
      | %<ID>
      | %<Vbase>V
      | %<VLF>pu
      | %<angleLF>deg.
      | %<Name>
  bus156 : powerlib/Measurements/Load Flow Bus  LConnTagsString=a  Phases=single  Connectors=on one side  ID=bus156  Vbase=220000  Vref=1  Vangle=0  VLF=1  VLFb=1  VLFc=1  angleLF=0  angleLFb=0  angleLFc=0
      settings: AttributesFormatString=|
      | %<ID>
      | %<Vbase>V
      | %<VLF>pu
      | %<angleLF>deg.
      | %<Name>
  bus157 : powerlib/Measurements/Load Flow Bus  LConnTagsString=a  Phases=single  Connectors=on one side  ID=bus157  Vbase=220000  Vref=1  Vangle=0  VLF=1  VLFb=1  VLFc=1  angleLF=0  angleLFb=0  angleLFc=0
      settings: AttributesFormatString=|
      | %<ID>
      | %<Vbase>V
      | %<VLF>pu
      | %<angleLF>deg.
      | %<Name>
  bus158 : powerlib/Measurements/Load Flow Bus  LConnTagsString=a  Phases=single  Connectors=on one side  ID=bus158  Vbase=220000  Vref=1  Vangle=0  VLF=1  VLFb=1  VLFc=1  angleLF=0  angleLFb=0  angleLFc=0
      settings: AttributesFormatString=|
      | %<ID>
      | %<Vbase>V
      | %<VLF>pu
      | %<angleLF>deg.
      | %<Name>
  bus159 : powerlib/Measurements/Load Flow Bus  LConnTagsString=a  Phases=single  Connectors=on one side  ID=bus159  Vbase=220000  Vref=1  Vangle=0  VLF=1  VLFb=1  VLFc=1  angleLF=0  angleLFb=0  angleLFc=0
      settings: AttributesFormatString=|
      | %<ID>
      | %<Vbase>V
      | %<VLF>pu
      | %<angleLF>deg.
      | %<Name>
  bus16 : powerlib/Measurements/Load Flow Bus  LConnTagsString=a  Phases=single  Connectors=on one side  ID=bus16  Vbase=220000  Vref=1  Vangle=0  VLF=1  VLFb=1  VLFc=1  angleLF=0  angleLFb=0  angleLFc=0
      settings: AttributesFormatString=|
      | %<ID>
      | %<Vbase>V
      | %<VLF>pu
      | %<angleLF>deg.
      | %<Name>
  bus160 : powerlib/Measurements/Load Flow Bus  LConnTagsString=a  Phases=single  Connectors=on one side  ID=bus160  Vbase=15000  Vref=1  Vangle=0  VLF=1  VLFb=1  VLFc=1  angleLF=0  angleLFb=0  angleLFc=0
      settings: AttributesFormatString=|
      | %<ID>
      | %<Vbase>V
      | %<VLF>pu
      | %<angleLF>deg.
      | %<Name>
  bus161 : powerlib/Measurements/Load Flow Bus  LConnTagsString=a  Phases=single  Connectors=on one side  ID=bus161  Vbase=220000  Vref=1  Vangle=0  VLF=1  VLFb=1  VLFc=1  angleLF=0  angleLFb=0  angleLFc=0
      settings: AttributesFormatString=|
      | %<ID>
      | %<Vbase>V
      | %<VLF>pu
      | %<angleLF>deg.
      | %<Name>
  bus162 : powerlib/Measurements/Load Flow Bus  LConnTagsString=a  Phases=single  Connectors=on one side  ID=bus162  Vbase=220000  Vref=1  Vangle=0  VLF=1  VLFb=1  VLFc=1  angleLF=0  angleLFb=0  angleLFc=0
      settings: AttributesFormatString=|
      | %<ID>
      | %<Vbase>V
      | %<VLF>pu
      | %<angleLF>deg.
      | %<Name>
  bus163 : powerlib/Measurements/Load Flow Bus  LConnTagsString=a  Phases=single  Connectors=on one side  ID=bus163  Vbase=220000  Vref=1  Vangle=0  VLF=1  VLFb=1  VLFc=1  angleLF=0  angleLFb=0  angleLFc=0
      settings: AttributesFormatString=|
      | %<ID>
      | %<Vbase>V
      | %<VLF>pu
      | %<angleLF>deg.
      | %<Name>
  bus164 : powerlib/Measurements/Load Flow Bus  LConnTagsString=a  Phases=single  Connectors=on one side  ID=bus164  Vbase=220000  Vref=1  Vangle=0  VLF=1  VLFb=1  VLFc=1  angleLF=0  angleLFb=0  angleLFc=0
      settings: AttributesFormatString=|
      | %<ID>
      | %<Vbase>V
      | %<VLF>pu
      | %<angleLF>deg.
      | %<Name>
  bus165 : powerlib/Measurements/Load Flow Bus  LConnTagsString=a  Phases=single  Connectors=on one side  ID=bus165  Vbase=220000  Vref=1  Vangle=0  VLF=1  VLFb=1  VLFc=1  angleLF=0  angleLFb=0  angleLFc=0
      settings: AttributesFormatString=|
      | %<ID>
      | %<Vbase>V
      | %<VLF>pu
      | %<angleLF>deg.
      | %<Name>
  bus166 : powerlib/Measurements/Load Flow Bus  LConnTagsString=a  Phases=single  Connectors=on one side  ID=bus166  Vbase=380000  Vref=1  Vangle=0  VLF=1  VLFb=1  VLFc=1  angleLF=0  angleLFb=0  angleLFc=0
      settings: AttributesFormatString=|
      | %<ID>
      | %<Vbase>V
      | %<VLF>pu
      | %<angleLF>deg.
      | %<Name>
  bus167 : powerlib/Measurements/Load Flow Bus  LConnTagsString=a  Phases=single  Connectors=on one side  ID=bus167  Vbase=220000  Vref=1  Vangle=0  VLF=1  VLFb=1  VLFc=1  angleLF=0  angleLFb=0  angleLFc=0
      settings: AttributesFormatString=|
      | %<ID>
      | %<Vbase>V
      | %<VLF>pu
      | %<angleLF>deg.
      | %<Name>
  bus168 : powerlib/Measurements/Load Flow Bus  LConnTagsString=a  Phases=single  Connectors=on one side  ID=bus168  Vbase=220000  Vref=1  Vangle=0  VLF=1  VLFb=1  VLFc=1  angleLF=0  angleLFb=0  angleLFc=0
      settings: AttributesFormatString=|
      | %<ID>
      | %<Vbase>V
      | %<VLF>pu
      | %<angleLF>deg.
      | %<Name>
  bus169 : powerlib/Measurements/Load Flow Bus  LConnTagsString=a  Phases=single  Connectors=on one side  ID=bus169  Vbase=220000  Vref=1  Vangle=0  VLF=1  VLFb=1  VLFc=1  angleLF=0  angleLFb=0  angleLFc=0
      settings: AttributesFormatString=|
      | %<ID>
      | %<Vbase>V
      | %<VLF>pu
      | %<angleLF>deg.
      | %<Name>
  bus17 : powerlib/Measurements/Load Flow Bus  LConnTagsString=a  Phases=single  Connectors=on one side  ID=bus17  Vbase=220000  Vref=1  Vangle=0  VLF=1  VLFb=1  VLFc=1  angleLF=0  angleLFb=0  angleLFc=0
      settings: AttributesFormatString=|
      | %<ID>
      | %<Vbase>V
      | %<VLF>pu
      | %<angleLF>deg.
      | %<Name>
  bus170 : powerlib/Measurements/Load Flow Bus  LConnTagsString=a  Phases=single  Connectors=on one side  ID=bus170  Vbase=220000  Vref=1  Vangle=0  VLF=1  VLFb=1  VLFc=1  angleLF=0  angleLFb=0  angleLFc=0
      settings: AttributesFormatString=|
      | %<ID>
      | %<Vbase>V
      | %<VLF>pu
      | %<angleLF>deg.
      | %<Name>
  bus171 : powerlib/Measurements/Load Flow Bus  LConnTagsString=a  Phases=single  Connectors=on one side  ID=bus171  Vbase=220000  Vref=1  Vangle=0  VLF=1  VLFb=1  VLFc=1  angleLF=0  angleLFb=0  angleLFc=0
      settings: AttributesFormatString=|
      | %<ID>
      | %<Vbase>V
      | %<VLF>pu
      | %<angleLF>deg.
      | %<Name>
  bus172 : powerlib/Measurements/Load Flow Bus  LConnTagsString=a  Phases=single  Connectors=on one side  ID=bus172  Vbase=220000  Vref=1  Vangle=0  VLF=1  VLFb=1  VLFc=1  angleLF=0  angleLFb=0  angleLFc=0
      settings: AttributesFormatString=|
      | %<ID>
      | %<Vbase>V
      | %<VLF>pu
      | %<angleLF>deg.
      | %<Name>
  bus173 : powerlib/Measurements/Load Flow Bus  LConnTagsString=a  Phases=single  Connectors=on one side  ID=bus173  Vbase=380000  Vref=1  Vangle=0  VLF=1  VLFb=1  VLFc=1  angleLF=0  angleLFb=0  angleLFc=0
      settings: AttributesFormatString=|
      | %<ID>
      | %<Vbase>V
      | %<VLF>pu
      | %<angleLF>deg.
      | %<Name>
  bus174 : powerlib/Measurements/Load Flow Bus  LConnTagsString=a  Phases=single  Connectors=on one side  ID=bus174  Vbase=220000  Vref=1  Vangle=0  VLF=1  VLFb=1  VLFc=1  angleLF=0  angleLFb=0  angleLFc=0
      settings: AttributesFormatString=|
      | %<ID>
      | %<Vbase>V
      | %<VLF>pu
      | %<angleLF>deg.
      | %<Name>
  bus175 : powerlib/Measurements/Load Flow Bus  LConnTagsString=a  Phases=single  Connectors=on one side  ID=bus175  Vbase=220000  Vref=1  Vangle=0  VLF=1  VLFb=1  VLFc=1  angleLF=0  angleLFb=0  angleLFc=0
      settings: AttributesFormatString=|
      | %<ID>
      | %<Vbase>V
      | %<VLF>pu
      | %<angleLF>deg.
      | %<Name>
  bus176 : powerlib/Measurements/Load Flow Bus  LConnTagsString=a  Phases=single  Connectors=on one side  ID=bus176  Vbase=220000  Vref=1  Vangle=0  VLF=1  VLFb=1  VLFc=1  angleLF=0  angleLFb=0  angleLFc=0
      settings: AttributesFormatString=|
      | %<ID>
      | %<Vbase>V
      | %<VLF>pu
      | %<angleLF>deg.
      | %<Name>
  bus177 : powerlib/Measurements/Load Flow Bus  LConnTagsString=a  Phases=single  Connectors=on one side  ID=bus177  Vbase=220000  Vref=1  Vangle=0  VLF=1  VLFb=1  VLFc=1  angleLF=0  angleLFb=0  angleLFc=0
      settings: AttributesFormatString=|
      | %<ID>
      | %<Vbase>V
      | %<VLF>pu
      | %<angleLF>deg.
      | %<Name>
  bus178 : powerlib/Measurements/Load Flow Bus  LConnTagsString=a  Phases=single  Connectors=on one side  ID=bus178  Vbase=220000  Vref=1  Vangle=0  VLF=1  VLFb=1  VLFc=1  angleLF=0  angleLFb=0  angleLFc=0
      settings: AttributesFormatString=|
      | %<ID>
      | %<Vbase>V
      | %<VLF>pu
      | %<angleLF>deg.
      | %<Name>
  bus179 : powerlib/Measurements/Load Flow Bus  LConnTagsString=a  Phases=single  Connectors=on one side  ID=bus179  Vbase=220000  Vref=1  Vangle=0  VLF=1  VLFb=1  VLFc=1  angleLF=0  angleLFb=0  angleLFc=0
      settings: AttributesFormatString=|
      | %<ID>
      | %<Vbase>V
      | %<VLF>pu
      | %<angleLF>deg.
      | %<Name>
  bus18 : powerlib/Measurements/Load Flow Bus  LConnTagsString=a  Phases=single  Connectors=on one side  ID=bus18  Vbase=220000  Vref=1  Vangle=0  VLF=1  VLFb=1  VLFc=1  angleLF=0  angleLFb=0  angleLFc=0
      settings: AttributesFormatString=|
      | %<ID>
      | %<Vbase>V
      | %<VLF>pu
      | %<angleLF>deg.
      | %<Name>
  bus180 : powerlib/Measurements/Load Flow Bus  LConnTagsString=a  Phases=single  Connectors=on one side  ID=bus180  Vbase=220000  Vref=1  Vangle=0  VLF=1  VLFb=1  VLFc=1  angleLF=0  angleLFb=0  angleLFc=0
      settings: AttributesFormatString=|
      | %<ID>
      | %<Vbase>V
      | %<VLF>pu
      | %<angleLF>deg.
      | %<Name>
  bus181 : powerlib/Measurements/Load Flow Bus  LConnTagsString=a  Phases=single  Connectors=on one side  ID=bus181  Vbase=220000  Vref=1  Vangle=0  VLF=1  VLFb=1  VLFc=1  angleLF=0  angleLFb=0  angleLFc=0
      settings: AttributesFormatString=|
      | %<ID>
      | %<Vbase>V
      | %<VLF>pu
      | %<angleLF>deg.
      | %<Name>
  bus182 : powerlib/Measurements/Load Flow Bus  LConnTagsString=a  Phases=single  Connectors=on one side  ID=bus182  Vbase=220000  Vref=1  Vangle=0  VLF=1  VLFb=1  VLFc=1  angleLF=0  angleLFb=0  angleLFc=0
      settings: AttributesFormatString=|
      | %<ID>
      | %<Vbase>V
      | %<VLF>pu
      | %<angleLF>deg.
      | %<Name>
  bus183 : powerlib/Measurements/Load Flow Bus  LConnTagsString=a  Phases=single  Connectors=on one side  ID=bus183  Vbase=220000  Vref=1  Vangle=0  VLF=1  VLFb=1  VLFc=1  angleLF=0  angleLFb=0  angleLFc=0
      settings: AttributesFormatString=|
      | %<ID>
      | %<Vbase>V
      | %<VLF>pu
      | %<angleLF>deg.
      | %<Name>
  bus184 : powerlib/Measurements/Load Flow Bus  LConnTagsString=a  Phases=single  Connectors=on one side  ID=bus184  Vbase=380000  Vref=1  Vangle=0  VLF=1  VLFb=1  VLFc=1  angleLF=0  angleLFb=0  angleLFc=0
      settings: AttributesFormatString=|
      | %<ID>
      | %<Vbase>V
      | %<VLF>pu
      | %<angleLF>deg.
      | %<Name>
  bus185 : powerlib/Measurements/Load Flow Bus  LConnTagsString=a  Phases=single  Connectors=on one side  ID=bus185  Vbase=380000  Vref=1  Vangle=0  VLF=1  VLFb=1  VLFc=1  angleLF=0  angleLFb=0  angleLFc=0
      settings: AttributesFormatString=|
      | %<ID>
      | %<Vbase>V
      | %<VLF>pu
      | %<angleLF>deg.
      | %<Name>
  bus186 : powerlib/Measurements/Load Flow Bus  LConnTagsString=a  Phases=single  Connectors=on one side  ID=bus186  Vbase=220000  Vref=1  Vangle=0  VLF=1  VLFb=1  VLFc=1  angleLF=0  angleLFb=0  angleLFc=0
      settings: AttributesFormatString=|
      | %<ID>
      | %<Vbase>V
      | %<VLF>pu
      | %<angleLF>deg.
      | %<Name>
  bus187 : powerlib/Measurements/Load Flow Bus  LConnTagsString=a  Phases=single  Connectors=on one side  ID=bus187  Vbase=220000  Vref=1  Vangle=0  VLF=1  VLFb=1  VLFc=1  angleLF=0  angleLFb=0  angleLFc=0
      settings: AttributesFormatString=|
      | %<ID>
      | %<Vbase>V
      | %<VLF>pu
      | %<angleLF>deg.
      | %<Name>
  bus188 : powerlib/Measurements/Load Flow Bus  LConnTagsString=a  Phases=single  Connectors=on one side  ID=bus188  Vbase=220000  Vref=1  Vangle=0  VLF=1  VLFb=1  VLFc=1  angleLF=0  angleLFb=0  angleLFc=0
      settings: AttributesFormatString=|
      | %<ID>
      | %<Vbase>V
      | %<VLF>pu
      | %<angleLF>deg.
      | %<Name>
  bus189 : powerlib/Measurements/Load Flow Bus  LConnTagsString=a  Phases=single  Connectors=on one side  ID=bus189  Vbase=220000  Vref=1  Vangle=0  VLF=1  VLFb=1  VLFc=1  angleLF=0  angleLFb=0  angleLFc=0
      settings: AttributesFormatString=|
      | %<ID>
      | %<Vbase>V
      | %<VLF>pu
      | %<angleLF>deg.
      | %<Name>
  bus19 : powerlib/Measurements/Load Flow Bus  LConnTagsString=a  Phases=single  Connectors=on one side  ID=bus19  Vbase=220000  Vref=1  Vangle=0  VLF=1  VLFb=1  VLFc=1  angleLF=0  angleLFb=0  angleLFc=0
      settings: AttributesFormatString=|
      | %<ID>
      | %<Vbase>V
      | %<VLF>pu
      | %<angleLF>deg.
      | %<Name>
  bus190 : powerlib/Measurements/Load Flow Bus  LConnTagsString=a  Phases=single  Connectors=on one side  ID=bus190  Vbase=220000  Vref=1  Vangle=0  VLF=1  VLFb=1  VLFc=1  angleLF=0  angleLFb=0  angleLFc=0
      settings: AttributesFormatString=|
      | %<ID>
      | %<Vbase>V
      | %<VLF>pu
      | %<angleLF>deg.
      | %<Name>
  bus191 : powerlib/Measurements/Load Flow Bus  LConnTagsString=a  Phases=single  Connectors=on one side  ID=bus191  Vbase=220000  Vref=1  Vangle=0  VLF=1  VLFb=1  VLFc=1  angleLF=0  angleLFb=0  angleLFc=0
      settings: AttributesFormatString=|
      | %<ID>
      | %<Vbase>V
      | %<VLF>pu
      | %<angleLF>deg.
      | %<Name>
  bus192 : powerlib/Measurements/Load Flow Bus  LConnTagsString=a  Phases=single  Connectors=on one side  ID=bus192  Vbase=220000  Vref=1  Vangle=0  VLF=1  VLFb=1  VLFc=1  angleLF=0  angleLFb=0  angleLFc=0
      settings: AttributesFormatString=|
      | %<ID>
      | %<Vbase>V
      | %<VLF>pu
      | %<angleLF>deg.
      | %<Name>
  bus2 : powerlib/Measurements/Load Flow Bus  LConnTagsString=a  Phases=single  Connectors=on one side  ID=bus2  Vbase=220000  Vref=1  Vangle=0  VLF=1  VLFb=1  VLFc=1  angleLF=0  angleLFb=0  angleLFc=0
      settings: AttributesFormatString=|
      | %<ID>
      | %<Vbase>V
      | %<VLF>pu
      | %<angleLF>deg.
      | %<Name>
  bus20 : powerlib/Measurements/Load Flow Bus  LConnTagsString=a  Phases=single  Connectors=on one side  ID=bus20  Vbase=380000  Vref=1  Vangle=0  VLF=1  VLFb=1  VLFc=1  angleLF=0  angleLFb=0  angleLFc=0
      settings: AttributesFormatString=|
      | %<ID>
      | %<Vbase>V
      | %<VLF>pu
      | %<angleLF>deg.
      | %<Name>
  bus21 : powerlib/Measurements/Load Flow Bus  LConnTagsString=a  Phases=single  Connectors=on one side  ID=bus21  Vbase=380000  Vref=1  Vangle=0  VLF=1  VLFb=1  VLFc=1  angleLF=0  angleLFb=0  angleLFc=0
      settings: AttributesFormatString=|
      | %<ID>
      | %<Vbase>V
      | %<VLF>pu
      | %<angleLF>deg.
      | %<Name>
  bus22 : powerlib/Measurements/Load Flow Bus  LConnTagsString=a  Phases=single  Connectors=on one side  ID=bus22  Vbase=220000  Vref=1  Vangle=0  VLF=1  VLFb=1  VLFc=1  angleLF=0  angleLFb=0  angleLFc=0
      settings: AttributesFormatString=|
      | %<ID>
      | %<Vbase>V
      | %<VLF>pu
      | %<angleLF>deg.
      | %<Name>
  bus23 : powerlib/Measurements/Load Flow Bus  LConnTagsString=a  Phases=single  Connectors=on one side  ID=bus23  Vbase=220000  Vref=1  Vangle=0  VLF=1  VLFb=1  VLFc=1  angleLF=0  angleLFb=0  angleLFc=0
      settings: AttributesFormatString=|
      | %<ID>
      | %<Vbase>V
      | %<VLF>pu
      | %<angleLF>deg.
      | %<Name>
  bus24 : powerlib/Measurements/Load Flow Bus  LConnTagsString=a  Phases=single  Connectors=on one side  ID=bus24  Vbase=380000  Vref=1  Vangle=0  VLF=1  VLFb=1  VLFc=1  angleLF=0  angleLFb=0  angleLFc=0
      settings: AttributesFormatString=|
      | %<ID>
      | %<Vbase>V
      | %<VLF>pu
      | %<angleLF>deg.
      | %<Name>
  bus25 : powerlib/Measurements/Load Flow Bus  LConnTagsString=a  Phases=single  Connectors=on one side  ID=bus25  Vbase=220000  Vref=1  Vangle=0  VLF=1  VLFb=1  VLFc=1  angleLF=0  angleLFb=0  angleLFc=0
      settings: AttributesFormatString=|
      | %<ID>
      | %<Vbase>V
      | %<VLF>pu
      | %<angleLF>deg.
      | %<Name>
  bus26 : powerlib/Measurements/Load Flow Bus  LConnTagsString=a  Phases=single  Connectors=on one side  ID=bus26  Vbase=220000  Vref=1  Vangle=0  VLF=1  VLFb=1  VLFc=1  angleLF=0  angleLFb=0  angleLFc=0
      settings: AttributesFormatString=|
      | %<ID>
      | %<Vbase>V
      | %<VLF>pu
      | %<angleLF>deg.
      | %<Name>
  bus27 : powerlib/Measurements/Load Flow Bus  LConnTagsString=a  Phases=single  Connectors=on one side  ID=bus27  Vbase=220000  Vref=1  Vangle=0  VLF=1  VLFb=1  VLFc=1  angleLF=0  angleLFb=0  angleLFc=0
      settings: AttributesFormatString=|
      | %<ID>
      | %<Vbase>V
      | %<VLF>pu
      | %<angleLF>deg.
      | %<Name>
  bus28 : powerlib/Measurements/Load Flow Bus  LConnTagsString=a  Phases=single  Connectors=on one side  ID=bus28  Vbase=220000  Vref=1  Vangle=0  VLF=1  VLFb=1  VLFc=1  angleLF=0  angleLFb=0  angleLFc=0
      settings: AttributesFormatString=|
      | %<ID>
      | %<Vbase>V
      | %<VLF>pu
      | %<angleLF>deg.
      | %<Name>
  bus29 : powerlib/Measurements/Load Flow Bus  LConnTagsString=a  Phases=single  Connectors=on one side  ID=bus29  Vbase=220000  Vref=1  Vangle=0  VLF=1  VLFb=1  VLFc=1  angleLF=0  angleLFb=0  angleLFc=0
      settings: AttributesFormatString=|
      | %<ID>
      | %<Vbase>V
      | %<VLF>pu
      | %<angleLF>deg.
      | %<Name>
  bus3 : powerlib/Measurements/Load Flow Bus  LConnTagsString=a  Phases=single  Connectors=on one side  ID=bus3  Vbase=380000  Vref=1  Vangle=0  VLF=1  VLFb=1  VLFc=1  angleLF=0  angleLFb=0  angleLFc=0
      settings: AttributesFormatString=|
      | %<ID>
      | %<Vbase>V
      | %<VLF>pu
      | %<angleLF>deg.
      | %<Name>
  bus30 : powerlib/Measurements/Load Flow Bus  LConnTagsString=a  Phases=single  Connectors=on one side  ID=bus30  Vbase=220000  Vref=1  Vangle=0  VLF=1  VLFb=1  VLFc=1  angleLF=0  angleLFb=0  angleLFc=0
      settings: AttributesFormatString=|
      | %<ID>
      | %<Vbase>V
      | %<VLF>pu
      | %<angleLF>deg.
      | %<Name>
  bus31 : powerlib/Measurements/Load Flow Bus  LConnTagsString=a  Phases=single  Connectors=on one side  ID=bus31  Vbase=220000  Vref=1  Vangle=0  VLF=1  VLFb=1  VLFc=1  angleLF=0  angleLFb=0  angleLFc=0
      settings: AttributesFormatString=|
      | %<ID>
      | %<Vbase>V
      | %<VLF>pu
      | %<angleLF>deg.
      | %<Name>
  bus32 : powerlib/Measurements/Load Flow Bus  LConnTagsString=a  Phases=single  Connectors=on one side  ID=bus32  Vbase=380000  Vref=1  Vangle=0  VLF=1  VLFb=1  VLFc=1  angleLF=0  angleLFb=0  angleLFc=0
      settings: AttributesFormatString=|
      | %<ID>
      | %<Vbase>V
      | %<VLF>pu
      | %<angleLF>deg.
      | %<Name>
  bus33 : powerlib/Measurements/Load Flow Bus  LConnTagsString=a  Phases=single  Connectors=on one side  ID=bus33  Vbase=380000  Vref=1  Vangle=0  VLF=1  VLFb=1  VLFc=1  angleLF=0  angleLFb=0  angleLFc=0
      settings: AttributesFormatString=|
      | %<ID>
      | %<Vbase>V
      | %<VLF>pu
      | %<angleLF>deg.
      | %<Name>
  bus34 : powerlib/Measurements/Load Flow Bus  LConnTagsString=a  Phases=single  Connectors=on one side  ID=bus34  Vbase=380000  Vref=1  Vangle=0  VLF=1  VLFb=1  VLFc=1  angleLF=0  angleLFb=0  angleLFc=0
      settings: AttributesFormatString=|
      | %<ID>
      | %<Vbase>V
      | %<VLF>pu
      | %<angleLF>deg.
      | %<Name>
  bus35 : powerlib/Measurements/Load Flow Bus  LConnTagsString=a  Phases=single  Connectors=on one side  ID=bus35  Vbase=220000  Vref=1  Vangle=0  VLF=1  VLFb=1  VLFc=1  angleLF=0  angleLFb=0  angleLFc=0
      settings: AttributesFormatString=|
      | %<ID>
      | %<Vbase>V
      | %<VLF>pu
      | %<angleLF>deg.
      | %<Name>
  bus36 : powerlib/Measurements/Load Flow Bus  LConnTagsString=a  Phases=single  Connectors=on one side  ID=bus36  Vbase=220000  Vref=1  Vangle=0  VLF=1  VLFb=1  VLFc=1  angleLF=0  angleLFb=0  angleLFc=0
      settings: AttributesFormatString=|
      | %<ID>
      | %<Vbase>V
      | %<VLF>pu
      | %<angleLF>deg.
      | %<Name>
  bus37 : powerlib/Measurements/Load Flow Bus  LConnTagsString=a  Phases=single  Connectors=on one side  ID=bus37  Vbase=220000  Vref=1  Vangle=0  VLF=1  VLFb=1  VLFc=1  angleLF=0  angleLFb=0  angleLFc=0
      settings: AttributesFormatString=|
      | %<ID>
      | %<Vbase>V
      | %<VLF>pu
      | %<angleLF>deg.
      | %<Name>
  bus38 : powerlib/Measurements/Load Flow Bus  LConnTagsString=a  Phases=single  Connectors=on one side  ID=bus38  Vbase=220000  Vref=1  Vangle=0  VLF=1  VLFb=1  VLFc=1  angleLF=0  angleLFb=0  angleLFc=0
      settings: AttributesFormatString=|
      | %<ID>
      | %<Vbase>V
      | %<VLF>pu
      | %<angleLF>deg.
      | %<Name>
  bus39 : powerlib/Measurements/Load Flow Bus  LConnTagsString=a  Phases=single  Connectors=on one side  ID=bus39  Vbase=220000  Vref=1  Vangle=0  VLF=1  VLFb=1  VLFc=1  angleLF=0  angleLFb=0  angleLFc=0
      settings: AttributesFormatString=|
      | %<ID>
      | %<Vbase>V
      | %<VLF>pu
      | %<angleLF>deg.
      | %<Name>
  bus4 : powerlib/Measurements/Load Flow Bus  LConnTagsString=a  Phases=single  Connectors=on one side  ID=bus4  Vbase=380000  Vref=1  Vangle=0  VLF=1  VLFb=1  VLFc=1  angleLF=0  angleLFb=0  angleLFc=0
      settings: AttributesFormatString=|
      | %<ID>
      | %<Vbase>V
      | %<VLF>pu
      | %<angleLF>deg.
      | %<Name>
  bus40 : powerlib/Measurements/Load Flow Bus  LConnTagsString=a  Phases=single  Connectors=on one side  ID=bus40  Vbase=220000  Vref=1  Vangle=0  VLF=1  VLFb=1  VLFc=1  angleLF=0  angleLFb=0  angleLFc=0
      settings: AttributesFormatString=|
      | %<ID>
      | %<Vbase>V
      | %<VLF>pu
      | %<angleLF>deg.
      | %<Name>
  bus41 : powerlib/Measurements/Load Flow Bus  LConnTagsString=a  Phases=single  Connectors=on one side  ID=bus41  Vbase=220000  Vref=1  Vangle=0  VLF=1  VLFb=1  VLFc=1  angleLF=0  angleLFb=0  angleLFc=0
      settings: AttributesFormatString=|
      | %<ID>
      | %<Vbase>V
      | %<VLF>pu
      | %<angleLF>deg.
      | %<Name>
  bus42 : powerlib/Measurements/Load Flow Bus  LConnTagsString=a  Phases=single  Connectors=on one side  ID=bus42  Vbase=220000  Vref=1  Vangle=0  VLF=1  VLFb=1  VLFc=1  angleLF=0  angleLFb=0  angleLFc=0
      settings: AttributesFormatString=|
      | %<ID>
      | %<Vbase>V
      | %<VLF>pu
      | %<angleLF>deg.
      | %<Name>
  bus43 : powerlib/Measurements/Load Flow Bus  LConnTagsString=a  Phases=single  Connectors=on one side  ID=bus43  Vbase=220000  Vref=1  Vangle=0  VLF=1  VLFb=1  VLFc=1  angleLF=0  angleLFb=0  angleLFc=0
      settings: AttributesFormatString=|
      | %<ID>
      | %<Vbase>V
      | %<VLF>pu
      | %<angleLF>deg.
      | %<Name>
  bus44 : powerlib/Measurements/Load Flow Bus  LConnTagsString=a  Phases=single  Connectors=on one side  ID=bus44  Vbase=220000  Vref=1  Vangle=0  VLF=1  VLFb=1  VLFc=1  angleLF=0  angleLFb=0  angleLFc=0
      settings: AttributesFormatString=|
      | %<ID>
      | %<Vbase>V
      | %<VLF>pu
      | %<angleLF>deg.
      | %<Name>
  bus45 : powerlib/Measurements/Load Flow Bus  LConnTagsString=a  Phases=single  Connectors=on one side  ID=bus45  Vbase=220000  Vref=1  Vangle=0  VLF=1  VLFb=1  VLFc=1  angleLF=0  angleLFb=0  angleLFc=0
      settings: AttributesFormatString=|
      | %<ID>
      | %<Vbase>V
      | %<VLF>pu
      | %<angleLF>deg.
      | %<Name>
  bus46 : powerlib/Measurements/Load Flow Bus  LConnTagsString=a  Phases=single  Connectors=on one side  ID=bus46  Vbase=220000  Vref=1  Vangle=0  VLF=1  VLFb=1  VLFc=1  angleLF=0  angleLFb=0  angleLFc=0
      settings: AttributesFormatString=|
      | %<ID>
      | %<Vbase>V
      | %<VLF>pu
      | %<angleLF>deg.
      | %<Name>
  bus47 : powerlib/Measurements/Load Flow Bus  LConnTagsString=a  Phases=single  Connectors=on one side  ID=bus47  Vbase=220000  Vref=1  Vangle=0  VLF=1  VLFb=1  VLFc=1  angleLF=0  angleLFb=0  angleLFc=0
      settings: AttributesFormatString=|
      | %<ID>
      | %<Vbase>V
      | %<VLF>pu
      | %<angleLF>deg.
      | %<Name>
  bus48 : powerlib/Measurements/Load Flow Bus  LConnTagsString=a  Phases=single  Connectors=on one side  ID=bus48  Vbase=380000  Vref=1  Vangle=0  VLF=1  VLFb=1  VLFc=1  angleLF=0  angleLFb=0  angleLFc=0
      settings: AttributesFormatString=|
      | %<ID>
      | %<Vbase>V
      | %<VLF>pu
      | %<angleLF>deg.
      | %<Name>
  bus49 : powerlib/Measurements/Load Flow Bus  LConnTagsString=a  Phases=single  Connectors=on one side  ID=bus49  Vbase=380000  Vref=1  Vangle=0  VLF=1  VLFb=1  VLFc=1  angleLF=0  angleLFb=0  angleLFc=0
      settings: AttributesFormatString=|
      | %<ID>
      | %<Vbase>V
      | %<VLF>pu
      | %<angleLF>deg.
      | %<Name>
  bus5 : powerlib/Measurements/Load Flow Bus  LConnTagsString=a  Phases=single  Connectors=on one side  ID=bus5  Vbase=380000  Vref=1  Vangle=0  VLF=1  VLFb=1  VLFc=1  angleLF=0  angleLFb=0  angleLFc=0
      settings: AttributesFormatString=|
      | %<ID>
      | %<Vbase>V
      | %<VLF>pu
      | %<angleLF>deg.
      | %<Name>
  bus50 : powerlib/Measurements/Load Flow Bus  LConnTagsString=a  Phases=single  Connectors=on one side  ID=bus50  Vbase=220000  Vref=1  Vangle=0  VLF=1  VLFb=1  VLFc=1  angleLF=0  angleLFb=0  angleLFc=0
      settings: AttributesFormatString=|
      | %<ID>
      | %<Vbase>V
      | %<VLF>pu
      | %<angleLF>deg.
      | %<Name>
  bus51 : powerlib/Measurements/Load Flow Bus  LConnTagsString=a  Phases=single  Connectors=on one side  ID=bus51  Vbase=220000  Vref=1  Vangle=0  VLF=1  VLFb=1  VLFc=1  angleLF=0  angleLFb=0  angleLFc=0
      settings: AttributesFormatString=|
      | %<ID>
      | %<Vbase>V
      | %<VLF>pu
      | %<angleLF>deg.
      | %<Name>
  bus52 : powerlib/Measurements/Load Flow Bus  LConnTagsString=a  Phases=single  Connectors=on one side  ID=bus52  Vbase=220000  Vref=1  Vangle=0  VLF=1  VLFb=1  VLFc=1  angleLF=0  angleLFb=0  angleLFc=0
      settings: AttributesFormatString=|
      | %<ID>
      | %<Vbase>V
      | %<VLF>pu
      | %<angleLF>deg.
      | %<Name>
  bus53 : powerlib/Measurements/Load Flow Bus  LConnTagsString=a  Phases=single  Connectors=on one side  ID=bus53  Vbase=220000  Vref=1  Vangle=0  VLF=1  VLFb=1  VLFc=1  angleLF=0  angleLFb=0  angleLFc=0
      settings: AttributesFormatString=|
      | %<ID>
      | %<Vbase>V
      | %<VLF>pu
      | %<angleLF>deg.
      | %<Name>
  bus54 : powerlib/Measurements/Load Flow Bus  LConnTagsString=a  Phases=single  Connectors=on one side  ID=bus54  Vbase=220000  Vref=1  Vangle=0  VLF=1  VLFb=1  VLFc=1  angleLF=0  angleLFb=0  angleLFc=0
      settings: AttributesFormatString=|
      | %<ID>
      | %<Vbase>V
      | %<VLF>pu
      | %<angleLF>deg.
      | %<Name>
  bus55 : powerlib/Measurements/Load Flow Bus  LConnTagsString=a  Phases=single  Connectors=on one side  ID=bus55  Vbase=380000  Vref=1  Vangle=0  VLF=1  VLFb=1  VLFc=1  angleLF=0  angleLFb=0  angleLFc=0
      settings: AttributesFormatString=|
      | %<ID>
      | %<Vbase>V
      | %<VLF>pu
      | %<angleLF>deg.
      | %<Name>
  bus56 : powerlib/Measurements/Load Flow Bus  LConnTagsString=a  Phases=single  Connectors=on one side  ID=bus56  Vbase=380000  Vref=1  Vangle=0  VLF=1  VLFb=1  VLFc=1  angleLF=0  angleLFb=0  angleLFc=0
      settings: AttributesFormatString=|
      | %<ID>
      | %<Vbase>V
      | %<VLF>pu
      | %<angleLF>deg.
      | %<Name>
  bus57 : powerlib/Measurements/Load Flow Bus  LConnTagsString=a  Phases=single  Connectors=on one side  ID=bus57  Vbase=380000  Vref=1  Vangle=0  VLF=1  VLFb=1  VLFc=1  angleLF=0  angleLFb=0  angleLFc=0
      settings: AttributesFormatString=|
      | %<ID>
      | %<Vbase>V
      | %<VLF>pu
      | %<angleLF>deg.
      | %<Name>
  bus58 : powerlib/Measurements/Load Flow Bus  LConnTagsString=a  Phases=single  Connectors=on one side  ID=bus58  Vbase=380000  Vref=1  Vangle=0  VLF=1  VLFb=1  VLFc=1  angleLF=0  angleLFb=0  angleLFc=0
      settings: AttributesFormatString=|
      | %<ID>
      | %<Vbase>V
      | %<VLF>pu
      | %<angleLF>deg.
      | %<Name>
  bus59 : powerlib/Measurements/Load Flow Bus  LConnTagsString=a  Phases=single  Connectors=on one side  ID=bus59  Vbase=380000  Vref=1  Vangle=0  VLF=1  VLFb=1  VLFc=1  angleLF=0  angleLFb=0  angleLFc=0
      settings: AttributesFormatString=|
      | %<ID>
      | %<Vbase>V
      | %<VLF>pu
      | %<angleLF>deg.
      | %<Name>
  bus6 : powerlib/Measurements/Load Flow Bus  LConnTagsString=a  Phases=single  Connectors=on one side  ID=bus6  Vbase=220000  Vref=1  Vangle=0  VLF=1  VLFb=1  VLFc=1  angleLF=0  angleLFb=0  angleLFc=0
      settings: AttributesFormatString=|
      | %<ID>
      | %<Vbase>V
      | %<VLF>pu
      | %<angleLF>deg.
      | %<Name>
  bus60 : powerlib/Measurements/Load Flow Bus  LConnTagsString=a  Phases=single  Connectors=on one side  ID=bus60  Vbase=220000  Vref=1  Vangle=0  VLF=1  VLFb=1  VLFc=1  angleLF=0  angleLFb=0  angleLFc=0
      settings: AttributesFormatString=|
      | %<ID>
      | %<Vbase>V
      | %<VLF>pu
      | %<angleLF>deg.
      | %<Name>
  bus61 : powerlib/Measurements/Load Flow Bus  LConnTagsString=a  Phases=single  Connectors=on one side  ID=bus61  Vbase=220000  Vref=1  Vangle=0  VLF=1  VLFb=1  VLFc=1  angleLF=0  angleLFb=0  angleLFc=0
      settings: AttributesFormatString=|
      | %<ID>
      | %<Vbase>V
      | %<VLF>pu
      | %<angleLF>deg.
      | %<Name>
  bus62 : powerlib/Measurements/Load Flow Bus  LConnTagsString=a  Phases=single  Connectors=on one side  ID=bus62  Vbase=220000  Vref=1  Vangle=0  VLF=1  VLFb=1  VLFc=1  angleLF=0  angleLFb=0  angleLFc=0
      settings: AttributesFormatString=|
      | %<ID>
      | %<Vbase>V
      | %<VLF>pu
      | %<angleLF>deg.
      | %<Name>
  bus63 : powerlib/Measurements/Load Flow Bus  LConnTagsString=a  Phases=single  Connectors=on one side  ID=bus63  Vbase=220000  Vref=1  Vangle=0  VLF=1  VLFb=1  VLFc=1  angleLF=0  angleLFb=0  angleLFc=0
      settings: AttributesFormatString=|
      | %<ID>
      | %<Vbase>V
      | %<VLF>pu
      | %<angleLF>deg.
      | %<Name>
  bus64 : powerlib/Measurements/Load Flow Bus  LConnTagsString=a  Phases=single  Connectors=on one side  ID=bus64  Vbase=220000  Vref=1  Vangle=0  VLF=1  VLFb=1  VLFc=1  angleLF=0  angleLFb=0  angleLFc=0
      settings: AttributesFormatString=|
      | %<ID>
      | %<Vbase>V
      | %<VLF>pu
      | %<angleLF>deg.
      | %<Name>
  bus65 : powerlib/Measurements/Load Flow Bus  LConnTagsString=a  Phases=single  Connectors=on one side  ID=bus65  Vbase=220000  Vref=1  Vangle=0  VLF=1  VLFb=1  VLFc=1  angleLF=0  angleLFb=0  angleLFc=0
      settings: AttributesFormatString=|
      | %<ID>
      | %<Vbase>V
      | %<VLF>pu
      | %<angleLF>deg.
      | %<Name>
  bus66 : powerlib/Measurements/Load Flow Bus  LConnTagsString=a  Phases=single  Connectors=on one side  ID=bus66  Vbase=220000  Vref=1  Vangle=0  VLF=1  VLFb=1  VLFc=1  angleLF=0  angleLFb=0  angleLFc=0
      settings: AttributesFormatString=|
      | %<ID>
      | %<Vbase>V
      | %<VLF>pu
      | %<angleLF>deg.
      | %<Name>
  bus67 : powerlib/Measurements/Load Flow Bus  LConnTagsString=a  Phases=single  Connectors=on one side  ID=bus67  Vbase=220000  Vref=1  Vangle=0  VLF=1  VLFb=1  VLFc=1  angleLF=0  angleLFb=0  angleLFc=0
      settings: AttributesFormatString=|
      | %<ID>
      | %<Vbase>V
      | %<VLF>pu
      | %<angleLF>deg.
      | %<Name>
  bus68 : powerlib/Measurements/Load Flow Bus  LConnTagsString=a  Phases=single  Connectors=on one side  ID=bus68  Vbase=220000  Vref=1  Vangle=0  VLF=1  VLFb=1  VLFc=1  angleLF=0  angleLFb=0  angleLFc=0
      settings: AttributesFormatString=|
      | %<ID>
      | %<Vbase>V
      | %<VLF>pu
      | %<angleLF>deg.
      | %<Name>
  bus69 : powerlib/Measurements/Load Flow Bus  LConnTagsString=a  Phases=single  Connectors=on one side  ID=bus69  Vbase=220000  Vref=1  Vangle=0  VLF=1  VLFb=1  VLFc=1  angleLF=0  angleLFb=0  angleLFc=0
      settings: AttributesFormatString=|
      | %<ID>
      | %<Vbase>V
      | %<VLF>pu
      | %<angleLF>deg.
      | %<Name>
  bus7 : powerlib/Measurements/Load Flow Bus  LConnTagsString=a  Phases=single  Connectors=on one side  ID=bus7  Vbase=220000  Vref=1  Vangle=0  VLF=1  VLFb=1  VLFc=1  angleLF=0  angleLFb=0  angleLFc=0
      settings: AttributesFormatString=|
      | %<ID>
      | %<Vbase>V
      | %<VLF>pu
      | %<angleLF>deg.
      | %<Name>
  bus70 : powerlib/Measurements/Load Flow Bus  LConnTagsString=a  Phases=single  Connectors=on one side  ID=bus70  Vbase=220000  Vref=1  Vangle=0  VLF=1  VLFb=1  VLFc=1  angleLF=0  angleLFb=0  angleLFc=0
      settings: AttributesFormatString=|
      | %<ID>
      | %<Vbase>V
      | %<VLF>pu
      | %<angleLF>deg.
      | %<Name>
  bus71 : powerlib/Measurements/Load Flow Bus  LConnTagsString=a  Phases=single  Connectors=on one side  ID=bus71  Vbase=380000  Vref=1  Vangle=0  VLF=1  VLFb=1  VLFc=1  angleLF=0  angleLFb=0  angleLFc=0
      settings: AttributesFormatString=|
      | %<ID>
      | %<Vbase>V
      | %<VLF>pu
      | %<angleLF>deg.
      | %<Name>
  bus72 : powerlib/Measurements/Load Flow Bus  LConnTagsString=a  Phases=single  Connectors=on one side  ID=bus72  Vbase=380000  Vref=1  Vangle=0  VLF=1  VLFb=1  VLFc=1  angleLF=0  angleLFb=0  angleLFc=0
      settings: AttributesFormatString=|
      | %<ID>
      | %<Vbase>V
      | %<VLF>pu
      | %<angleLF>deg.
      | %<Name>
  bus73 : powerlib/Measurements/Load Flow Bus  LConnTagsString=a  Phases=single  Connectors=on one side  ID=bus73  Vbase=380000  Vref=1  Vangle=0  VLF=1  VLFb=1  VLFc=1  angleLF=0  angleLFb=0  angleLFc=0
      settings: AttributesFormatString=|
      | %<ID>
      | %<Vbase>V
      | %<VLF>pu
      | %<angleLF>deg.
      | %<Name>
  bus74 : powerlib/Measurements/Load Flow Bus  LConnTagsString=a  Phases=single  Connectors=on one side  ID=bus74  Vbase=220000  Vref=1  Vangle=0  VLF=1  VLFb=1  VLFc=1  angleLF=0  angleLFb=0  angleLFc=0
      settings: AttributesFormatString=|
      | %<ID>
      | %<Vbase>V
      | %<VLF>pu
      | %<angleLF>deg.
      | %<Name>
  bus75 : powerlib/Measurements/Load Flow Bus  LConnTagsString=a  Phases=single  Connectors=on one side  ID=bus75  Vbase=220000  Vref=1  Vangle=0  VLF=1  VLFb=1  VLFc=1  angleLF=0  angleLFb=0  angleLFc=0
      settings: AttributesFormatString=|
      | %<ID>
      | %<Vbase>V
      | %<VLF>pu
      | %<angleLF>deg.
      | %<Name>
  bus76 : powerlib/Measurements/Load Flow Bus  LConnTagsString=a  Phases=single  Connectors=on one side  ID=bus76  Vbase=220000  Vref=1  Vangle=0  VLF=1  VLFb=1  VLFc=1  angleLF=0  angleLFb=0  angleLFc=0
      settings: AttributesFormatString=|
      | %<ID>
      | %<Vbase>V
      | %<VLF>pu
      | %<angleLF>deg.
      | %<Name>
  bus77 : powerlib/Measurements/Load Flow Bus  LConnTagsString=a  Phases=single  Connectors=on one side  ID=bus77  Vbase=220000  Vref=1  Vangle=0  VLF=1  VLFb=1  VLFc=1  angleLF=0  angleLFb=0  angleLFc=0
      settings: AttributesFormatString=|
      | %<ID>
      | %<Vbase>V
      | %<VLF>pu
      | %<angleLF>deg.
      | %<Name>
  bus78 : powerlib/Measurements/Load Flow Bus  LConnTagsString=a  Phases=single  Connectors=on one side  ID=bus78  Vbase=220000  Vref=1  Vangle=0  VLF=1  VLFb=1  VLFc=1  angleLF=0  angleLFb=0  angleLFc=0
      settings: AttributesFormatString=|
      | %<ID>
      | %<Vbase>V
      | %<VLF>pu
      | %<angleLF>deg.
      | %<Name>
  bus79 : powerlib/Measurements/Load Flow Bus  LConnTagsString=a  Phases=single  Connectors=on one side  ID=bus79  Vbase=220000  Vref=1  Vangle=0  VLF=1  VLFb=1  VLFc=1  angleLF=0  angleLFb=0  angleLFc=0
      settings: AttributesFormatString=|
      | %<ID>
      | %<Vbase>V
      | %<VLF>pu
      | %<angleLF>deg.
      | %<Name>
  bus8 : powerlib/Measurements/Load Flow Bus  LConnTagsString=a  Phases=single  Connectors=on one side  ID=bus8  Vbase=220000  Vref=1  Vangle=0  VLF=1  VLFb=1  VLFc=1  angleLF=0  angleLFb=0  angleLFc=0
      settings: AttributesFormatString=|
      | %<ID>
      | %<Vbase>V
      | %<VLF>pu
      | %<angleLF>deg.
      | %<Name>
  bus80 : powerlib/Measurements/Load Flow Bus  LConnTagsString=a  Phases=single  Connectors=on one side  ID=bus80  Vbase=220000  Vref=1  Vangle=0  VLF=1  VLFb=1  VLFc=1  angleLF=0  angleLFb=0  angleLFc=0
      settings: AttributesFormatString=|
      | %<ID>
      | %<Vbase>V
      | %<VLF>pu
      | %<angleLF>deg.
      | %<Name>
  bus81 : powerlib/Measurements/Load Flow Bus  LConnTagsString=a  Phases=single  Connectors=on one side  ID=bus81  Vbase=380000  Vref=1  Vangle=0  VLF=1  VLFb=1  VLFc=1  angleLF=0  angleLFb=0  angleLFc=0
      settings: AttributesFormatString=|
      | %<ID>
      | %<Vbase>V
      | %<VLF>pu
      | %<angleLF>deg.
      | %<Name>
  bus82 : powerlib/Measurements/Load Flow Bus  LConnTagsString=a  Phases=single  Connectors=on one side  ID=bus82  Vbase=380000  Vref=1  Vangle=0  VLF=1  VLFb=1  VLFc=1  angleLF=0  angleLFb=0  angleLFc=0
      settings: AttributesFormatString=|
      | %<ID>
      | %<Vbase>V
      | %<VLF>pu
      | %<angleLF>deg.
      | %<Name>
  bus83 : powerlib/Measurements/Load Flow Bus  LConnTagsString=a  Phases=single  Connectors=on one side  ID=bus83  Vbase=220000  Vref=1  Vangle=0  VLF=1  VLFb=1  VLFc=1  angleLF=0  angleLFb=0  angleLFc=0
      settings: AttributesFormatString=|
      | %<ID>
      | %<Vbase>V
      | %<VLF>pu
      | %<angleLF>deg.
      | %<Name>
  bus84 : powerlib/Measurements/Load Flow Bus  LConnTagsString=a  Phases=single  Connectors=on one side  ID=bus84  Vbase=220000  Vref=1  Vangle=0  VLF=1  VLFb=1  VLFc=1  angleLF=0  angleLFb=0  angleLFc=0
      settings: AttributesFormatString=|
      | %<ID>
      | %<Vbase>V
      | %<VLF>pu
      | %<angleLF>deg.
      | %<Name>
  bus85 : powerlib/Measurements/Load Flow Bus  LConnTagsString=a  Phases=single  Connectors=on one side  ID=bus85  Vbase=220000  Vref=1  Vangle=0  VLF=1  VLFb=1  VLFc=1  angleLF=0  angleLFb=0  angleLFc=0
      settings: AttributesFormatString=|
      | %<ID>
      | %<Vbase>V
      | %<VLF>pu
      | %<angleLF>deg.
      | %<Name>
  bus86 : powerlib/Measurements/Load Flow Bus  LConnTagsString=a  Phases=single  Connectors=on one side  ID=bus86  Vbase=220000  Vref=1  Vangle=0  VLF=1  VLFb=1  VLFc=1  angleLF=0  angleLFb=0  angleLFc=0
      settings: AttributesFormatString=|
      | %<ID>
      | %<Vbase>V
      | %<VLF>pu
      | %<angleLF>deg.
      | %<Name>
  bus87 : powerlib/Measurements/Load Flow Bus  LConnTagsString=a  Phases=single  Connectors=on one side  ID=bus87  Vbase=220000  Vref=1  Vangle=0  VLF=1  VLFb=1  VLFc=1  angleLF=0  angleLFb=0  angleLFc=0
      settings: AttributesFormatString=|
      | %<ID>
      | %<Vbase>V
      | %<VLF>pu
      | %<angleLF>deg.
      | %<Name>
  bus88 : powerlib/Measurements/Load Flow Bus  LConnTagsString=a  Phases=single  Connectors=on one side  ID=bus88  Vbase=220000  Vref=1  Vangle=0  VLF=1  VLFb=1  VLFc=1  angleLF=0  angleLFb=0  angleLFc=0
      settings: AttributesFormatString=|
      | %<ID>
      | %<Vbase>V
      | %<VLF>pu
      | %<angleLF>deg.
      | %<Name>
  bus89 : powerlib/Measurements/Load Flow Bus  LConnTagsString=a  Phases=single  Connectors=on one side  ID=bus89  Vbase=220000  Vref=1  Vangle=0  VLF=1  VLFb=1  VLFc=1  angleLF=0  angleLFb=0  angleLFc=0
      settings: AttributesFormatString=|
      | %<ID>
      | %<Vbase>V
      | %<VLF>pu
      | %<angleLF>deg.
      | %<Name>
  bus9 : powerlib/Measurements/Load Flow Bus  LConnTagsString=a  Phases=single  Connectors=on one side  ID=bus9  Vbase=220000  Vref=1  Vangle=0  VLF=1  VLFb=1  VLFc=1  angleLF=0  angleLFb=0  angleLFc=0
      settings: AttributesFormatString=|
      | %<ID>
      | %<Vbase>V
      | %<VLF>pu
      | %<angleLF>deg.
      | %<Name>
  bus90 : powerlib/Measurements/Load Flow Bus  LConnTagsString=a  Phases=single  Connectors=on one side  ID=bus90  Vbase=380000  Vref=1  Vangle=0  VLF=1  VLFb=1  VLFc=1  angleLF=0  angleLFb=0  angleLFc=0
      settings: AttributesFormatString=|
      | %<ID>
      | %<Vbase>V
      | %<VLF>pu
      | %<angleLF>deg.
      | %<Name>
  bus91 : powerlib/Measurements/Load Flow Bus  LConnTagsString=a  Phases=single  Connectors=on one side  ID=bus91  Vbase=220000  Vref=1  Vangle=0  VLF=1  VLFb=1  VLFc=1  angleLF=0  angleLFb=0  angleLFc=0
      settings: AttributesFormatString=|
      | %<ID>
      | %<Vbase>V
      | %<VLF>pu
      | %<angleLF>deg.
      | %<Name>
  bus92 : powerlib/Measurements/Load Flow Bus  LConnTagsString=a  Phases=single  Connectors=on one side  ID=bus92  Vbase=220000  Vref=1  Vangle=0  VLF=1  VLFb=1  VLFc=1  angleLF=0  angleLFb=0  angleLFc=0
      settings: AttributesFormatString=|
      | %<ID>
      | %<Vbase>V
      | %<VLF>pu
      | %<angleLF>deg.
      | %<Name>
  bus93 : powerlib/Measurements/Load Flow Bus  LConnTagsString=a  Phases=single  Connectors=on one side  ID=bus93  Vbase=220000  Vref=1  Vangle=0  VLF=1  VLFb=1  VLFc=1  angleLF=0  angleLFb=0  angleLFc=0
      settings: AttributesFormatString=|
      | %<ID>
      | %<Vbase>V
      | %<VLF>pu
      | %<angleLF>deg.
      | %<Name>
  bus94 : powerlib/Measurements/Load Flow Bus  LConnTagsString=a  Phases=single  Connectors=on one side  ID=bus94  Vbase=220000  Vref=1  Vangle=0  VLF=1  VLFb=1  VLFc=1  angleLF=0  angleLFb=0  angleLFc=0
      settings: AttributesFormatString=|
      | %<ID>
      | %<Vbase>V
      | %<VLF>pu
      | %<angleLF>deg.
      | %<Name>
  bus95 : powerlib/Measurements/Load Flow Bus  LConnTagsString=a  Phases=single  Connectors=on one side  ID=bus95  Vbase=220000  Vref=1  Vangle=0  VLF=1  VLFb=1  VLFc=1  angleLF=0  angleLFb=0  angleLFc=0
      settings: AttributesFormatString=|
      | %<ID>
      | %<Vbase>V
      | %<VLF>pu
      | %<angleLF>deg.
      | %<Name>
  bus96 : powerlib/Measurements/Load Flow Bus  LConnTagsString=a  Phases=single  Connectors=on one side  ID=bus96  Vbase=220000  Vref=1  Vangle=0  VLF=1  VLFb=1  VLFc=1  angleLF=0  angleLFb=0  angleLFc=0
      settings: AttributesFormatString=|
      | %<ID>
      | %<Vbase>V
      | %<VLF>pu
      | %<angleLF>deg.
      | %<Name>
  bus97 : powerlib/Measurements/Load Flow Bus  LConnTagsString=a  Phases=single  Connectors=on one side  ID=bus97  Vbase=380000  Vref=1  Vangle=0  VLF=1  VLFb=1  VLFc=1  angleLF=0  angleLFb=0  angleLFc=0
      settings: AttributesFormatString=|
      | %<ID>
      | %<Vbase>V
      | %<VLF>pu
      | %<angleLF>deg.
      | %<Name>
  bus98 : powerlib/Measurements/Load Flow Bus  LConnTagsString=a  Phases=single  Connectors=on one side  ID=bus98  Vbase=380000  Vref=1  Vangle=0  VLF=1  VLFb=1  VLFc=1  angleLF=0  angleLFb=0  angleLFc=0
      settings: AttributesFormatString=|
      | %<ID>
      | %<Vbase>V
      | %<VLF>pu
      | %<angleLF>deg.
      | %<Name>
  bus99 : powerlib/Measurements/Load Flow Bus  LConnTagsString=a  Phases=single  Connectors=on one side  ID=bus99  Vbase=380000  Vref=1  Vangle=0  VLF=1  VLFb=1  VLFc=1  angleLF=0  angleLFb=0  angleLFc=0
      settings: AttributesFormatString=|
      | %<ID>
      | %<Vbase>V
      | %<VLF>pu
      | %<angleLF>deg.
      | %<Name>
  powergui : powerlib/powergui  Priority=1  SimulationMode=Phasor  SolverType=Tustin/Backward Euler (TBE)  SampleTime=50e-6  frequency=50  SPID=off  DisableSnubberDevices=off  DisableRonSwitches=off  DisableVfSwitches=off  SwTol=0  DisplayEquations=off  Interpol=off  ExternalGateDelay=off  methode=off  Ts=10  FunctionMessages=off  echomessages=off  HookPort=off  EnableUseOfTLC=off  x0status=blocks  frequencyindice=50  Pbase=3000e6  ErrMax=0.0001  Iterations=50  UnitsV=V  UnitsW=W  buscounter=0  RestoreLinks=warning  ResistiveCurrentMeasurement=off  Frange=[0:2:500]  Ylog=off  Xlog=on  ShowGrid=off  save=off  variable=ZData  structure=0  ZoomFFT=off  StartTime=0.0  cycles=1  DisplayStyle=1  fundamental=60  FreqAxis=off  MaxFrequency=1000  frequencyindicesteady=1  RmsSteady=1  display=off
  connections:
  T_140873735__/LConn1 -- _CN_140873735_220000_CN_281800404_220000/LConn1
  T_140873735__/LConn2 -- _CN_140873735_220000_CN_281800404_220000/LConn2
  _CN_140873735_220000_CN_281800404_220000/LConn3 -- T_140873735__/LConn3 -- bus1/LConn1
  _CN_140873735_220000_CN_281800404_220000/RConn1 -- T_281800404__Umspannwerk_Avegno/LConn1 -- _CN_281803398_220000_CN_281800404_220000/LConn1 -- Centrale_Verbano___Avegno_CN_281810588_220000_CN_281800404_220000/LConn1
  _CN_140873735_220000_CN_281800404_220000/RConn2 -- T_281800404__Umspannwerk_Avegno/LConn2 -- _CN_281803398_220000_CN_281800404_220000/LConn2 -- Centrale_Verbano___Avegno_CN_281810588_220000_CN_281800404_220000/LConn2
  _CN_140873735_220000_CN_281800404_220000/RConn3 -- T_281800404__Umspannwerk_Avegno/LConn3 -- _CN_281803398_220000_CN_281800404_220000/LConn3 -- Centrale_Verbano___Avegno_CN_281810588_220000_CN_281800404_220000/LConn3 -- bus2/LConn1
  _CN_356292116_380000_CN_50319857_380000/LConn1 -- T_356292116__/LConn1 -- _CN_356292116_380000_CN_40639427_380000/LConn1
  _CN_356292116_380000_CN_50319857_380000/LConn2 -- T_356292116__/LConn2 -- _CN_356292116_380000_CN_40639427_380000/LConn2
  _CN_356292116_380000_CN_50319857_380000/LConn3 -- T_356292116__/LConn3 -- _CN_356292116_380000_CN_40639427_380000/LConn3 -- bus3/LConn1
  _CN_356292116_380000_CN_50319857_380000/RConn1 -- T_50319857_380000;220000_Laufenburg/LConn1 -- _CN_164850027_380000_CN_50319857_380000/LConn1 -- _CN_98648381_380000_CN_50319857_380000/LConn1 -- _CN_397960460_380000_CN_50319857_380000/LConn1 -- _CN_35840165_380000_CN_50319857_380000/LConn1
  _CN_356292116_380000_CN_50319857_380000/RConn2 -- T_50319857_380000;220000_Laufenburg/LConn2 -- _CN_164850027_380000_CN_50319857_380000/LConn2 -- _CN_98648381_380000_CN_50319857_380000/LConn2 -- _CN_397960460_380000_CN_50319857_380000/LConn2 -- _CN_35840165_380000_CN_50319857_380000/LConn2
  _CN_356292116_380000_CN_50319857_380000/RConn3 -- T_50319857_380000;220000_Laufenburg/LConn3 -- _CN_164850027_380000_CN_50319857_380000/LConn3 -- bus4/LConn1 -- _CN_98648381_380000_CN_50319857_380000/LConn3 -- _CN_397960460_380000_CN_50319857_380000/LConn3 -- _CN_35840165_380000_CN_50319857_380000/LConn3
  _CN_356292116_380000_CN_40639427_380000/RConn1 -- T_40639427__Gösgen/LConn1 -- _CN_40639427_380000_CN_35002638_380000/LConn1
  _CN_356292116_380000_CN_40639427_380000/RConn2 -- T_40639427__Gösgen/LConn2 -- _CN_40639427_380000_CN_35002638_380000/LConn2
  _CN_356292116_380000_CN_40639427_380000/RConn3 -- T_40639427__Gösgen/LConn3 -- _CN_40639427_380000_CN_35002638_380000/LConn3 -- bus5/LConn1
  _CN_356292116_220000_CN_30350721_220000/LConn1 -- T_356292116__/RConn4 -- _CN_356292116_220000_CN33394785/LConn1 -- _CN_356292116_220000_CN_146225999_220000/LConn1 -- _CN_356292116_220000_CN_35002638_220000/LConn1
  _CN_356292116_220000_CN_30350721_220000/LConn2 -- T_356292116__/RConn5 -- _CN_356292116_220000_CN33394785/LConn2 -- _CN_356292116_220000_CN_146225999_220000/LConn2 -- _CN_356292116_220000_CN_35002638_220000/LConn2
  _CN_356292116_220000_CN_30350721_220000/LConn3 -- T_356292116__/RConn6 -- _CN_356292116_220000_CN33394785/LConn3 -- _CN_356292116_220000_CN_146225999_220000/LConn3 -- _CN_356292116_220000_CN_35002638_220000/LConn3 -- bus6/LConn1
  _CN_356292116_220000_CN_30350721_220000/RConn1 -- T_30350721__Ormalingen/RConn1 -- _CN_30350721_220000_CN_27435934_220000/LConn1
  _CN_356292116_220000_CN_30350721_220000/RConn2 -- T_30350721__Ormalingen/RConn2 -- _CN_30350721_220000_CN_27435934_220000/LConn2
  _CN_356292116_220000_CN_30350721_220000/RConn3 -- T_30350721__Ormalingen/RConn3 -- _CN_30350721_220000_CN_27435934_220000/LConn3 -- bus7/LConn1
  G_33394785_Kernkraftwerk_Gösgen/RConn1 -- _CN_356292116_220000_CN33394785/RConn1
  G_33394785_Kernkraftwerk_Gösgen/RConn2 -- _CN_356292116_220000_CN33394785/RConn2
  _CN_356292116_220000_CN33394785/RConn3 -- G_33394785_Kernkraftwerk_Gösgen/RConn3 -- bus8/LConn1
  T_146225999__Sursee/LConn1 -- _CN_356292116_220000_CN_146225999_220000/RConn1
  T_146225999__Sursee/LConn2 -- _CN_356292116_220000_CN_146225999_220000/RConn2
  _CN_356292116_220000_CN_146225999_220000/RConn3 -- T_146225999__Sursee/LConn3 -- bus9/LConn1
  _CN_356292116_220000_CN_35002638_220000/RConn1 -- T_35002638__Mettlen/RConn1 -- _CN_35002638_220000_CN_164850030_220000/LConn1
  _CN_356292116_220000_CN_35002638_220000/RConn2 -- T_35002638__Mettlen/RConn2 -- _CN_35002638_220000_CN_164850030_220000/LConn2
  _CN_356292116_220000_CN_35002638_220000/RConn3 -- T_35002638__Mettlen/RConn3 -- _CN_35002638_220000_CN_164850030_220000/LConn3 -- bus10/LConn1
  _CN_26843160_220000_CN_147714395_220000/LConn1 -- T_26843160_220000_Weinfelden/LConn1 -- _CN_26843160_220000_CN_240575085_220000/LConn1 -- _CN_26843160_220000_CN_192677427_220000/LConn1 -- _CN_26843160_220000_CN_11282314_220000/LConn1 -- _CN_26843160_220000_CN_92798668_220000/LConn1
  _CN_26843160_220000_CN_147714395_220000/LConn2 -- T_26843160_220000_Weinfelden/LConn2 -- _CN_26843160_220000_CN_240575085_220000/LConn2 -- _CN_26843160_220000_CN_192677427_220000/LConn2 -- _CN_26843160_220000_CN_11282314_220000/LConn2 -- _CN_26843160_220000_CN_92798668_220000/LConn2
  _CN_26843160_220000_CN_147714395_220000/LConn3 -- T_26843160_220000_Weinfelden/LConn3 -- _CN_26843160_220000_CN_240575085_220000/LConn3 -- _CN_26843160_220000_CN_192677427_220000/LConn3 -- _CN_26843160_220000_CN_11282314_220000/LConn3 -- _CN_26843160_220000_CN_92798668_220000/LConn3 -- bus11/LConn1
  _CN_26843160_220000_CN_147714395_220000/RConn1 -- T_147714395__/RConn1 -- _CN_192677427_220000_CN_147714395_220000/LConn1 -- _CN_147714395_220000_CN_50561341_220000/LConn1 -- _CN_147714395_220000_CN_87281514_220000/LConn1
  _CN_26843160_220000_CN_147714395_220000/RConn2 -- T_147714395__/RConn2 -- _CN_192677427_220000_CN_147714395_220000/LConn2 -- _CN_147714395_220000_CN_50561341_220000/LConn2 -- _CN_147714395_220000_CN_87281514_220000/LConn2
  _CN_26843160_220000_CN_147714395_220000/RConn3 -- T_147714395__/RConn3 -- _CN_192677427_220000_CN_147714395_220000/LConn3 -- _CN_147714395_220000_CN_50561341_220000/LConn3 -- _CN_147714395_220000_CN_87281514_220000/LConn3 -- bus12/LConn1
  T_240575085_220000_Aathal/LConn1 -- _CN_26843160_220000_CN_240575085_220000/RConn1
  T_240575085_220000_Aathal/LConn2 -- _CN_26843160_220000_CN_240575085_220000/RConn2
  _CN_26843160_220000_CN_240575085_220000/RConn3 -- T_240575085_220000_Aathal/LConn3 -- bus13/LConn1
  _CN_26843160_220000_CN_192677427_220000/RConn1 -- T_192677427_380000;220000_Grynau/LConn1 -- _CN_192677427_220000_CN_92798668_220000/LConn1 -- _CN_192677427_220000_CN_147714395_220000/RConn1 -- _CN_192677427_220000_CN_365590455_220000/LConn1 -- _CN_192677427_220000_CN_210568055_220000/LConn1
  _CN_26843160_220000_CN_192677427_220000/RConn2 -- T_192677427_380000;220000_Grynau/LConn2 -- _CN_192677427_220000_CN_92798668_220000/LConn2 -- _CN_192677427_220000_CN_147714395_220000/RConn2 -- _CN_192677427_220000_CN_365590455_220000/LConn2 -- _CN_192677427_220000_CN_210568055_220000/LConn2
  _CN_26843160_220000_CN_192677427_220000/RConn3 -- T_192677427_380000;220000_Grynau/LConn3 -- _CN_192677427_220000_CN_92798668_220000/LConn3 -- _CN_192677427_220000_CN_147714395_220000/RConn3 -- _CN_192677427_220000_CN_365590455_220000/LConn3 -- bus14/LConn1 -- _CN_192677427_220000_CN_210568055_220000/LConn3
  _CN_26843160_220000_CN_11282314_220000/RConn1 -- T_11282314__Unterwerk_Fällanden/LConn1 -- _CN_11282314_220000_CN_193131937_220000/LConn1
  _CN_26843160_220000_CN_11282314_220000/RConn2 -- T_11282314__Unterwerk_Fällanden/LConn2 -- _CN_11282314_220000_CN_193131937_220000/LConn2
  _CN_26843160_220000_CN_11282314_220000/RConn3 -- T_11282314__Unterwerk_Fällanden/LConn3 -- _CN_11282314_220000_CN_193131937_220000/LConn3 -- bus15/LConn1
  _CN_26843160_220000_CN_92798668_220000/RConn1 -- T_92798668_220000_Winkeln/LConn1 -- Stoss_Süd;Falknis_CN_92798668_220000_CN_83861269_220000/LConn1 -- Stoss_Süd;Falknis_CN_92798668_220000_CN_92873516_220000/LConn1 -- _CN_192677427_220000_CN_92798668_220000/RConn1
  _CN_26843160_220000_CN_92798668_220000/RConn2 -- T_92798668_220000_Winkeln/LConn2 -- Stoss_Süd;Falknis_CN_92798668_220000_CN_83861269_220000/LConn2 -- Stoss_Süd;Falknis_CN_92798668_220000_CN_92873516_220000/LConn2 -- _CN_192677427_220000_CN_92798668_220000/RConn2
  _CN_26843160_220000_CN_92798668_220000/RConn3 -- T_92798668_220000_Winkeln/LConn3 -- Stoss_Süd;Falknis_CN_92798668_220000_CN_83861269_220000/LConn3 -- Stoss_Süd;Falknis_CN_92798668_220000_CN_92873516_220000/LConn3 -- bus16/LConn1 -- _CN_192677427_220000_CN_92798668_220000/RConn3
  _CN_71500123_220000_CN_365556107_220000/LConn1 -- T_71500123__Bonaduz/RConn1 -- _CN_71500123_220000_CN_211907009_220000/LConn1 -- _CN_71500123_220000_CN_210568055_220000/LConn1 -- _CN_71500123_220000_CN_36348118_220000/LConn1
  _CN_71500123_220000_CN_365556107_220000/LConn2 -- T_71500123__Bonaduz/RConn2 -- _CN_71500123_220000_CN_211907009_220000/LConn2 -- _CN_71500123_220000_CN_210568055_220000/LConn2 -- _CN_71500123_220000_CN_36348118_220000/LConn2
  _CN_71500123_220000_CN_365556107_220000/LConn3 -- T_71500123__Bonaduz/RConn3 -- _CN_71500123_220000_CN_211907009_220000/LConn3 -- bus17/LConn1 -- _CN_71500123_220000_CN_210568055_220000/LConn3 -- _CN_71500123_220000_CN_36348118_220000/LConn3
  T_365556107__Ilanz/LConn1 -- _CN_71500123_220000_CN_365556107_220000/RConn1
  T_365556107__Ilanz/LConn2 -- _CN_71500123_220000_CN_365556107_220000/RConn2
  _CN_71500123_220000_CN_365556107_220000/RConn3 -- T_365556107__Ilanz/LConn3 -- bus18/LConn1
  _CN_71500123_220000_CN_210568055_220000/RConn1 -- T_210568055__Schaltanlage_Tavanasa/RConn1 -- _CN_100662075_220000_CN_210568055_220000/LConn1 -- _CN_192677427_220000_CN_210568055_220000/RConn1
  _CN_71500123_220000_CN_210568055_220000/RConn2 -- T_210568055__Schaltanlage_Tavanasa/RConn2 -- _CN_100662075_220000_CN_210568055_220000/LConn2 -- _CN_192677427_220000_CN_210568055_220000/RConn2
  _CN_71500123_220000_CN_210568055_220000/RConn3 -- T_210568055__Schaltanlage_Tavanasa/RConn3 -- _CN_100662075_220000_CN_210568055_220000/LConn3 -- bus19/LConn1 -- _CN_192677427_220000_CN_210568055_220000/RConn3
  Bonaduz_CN_71500123_380000_CN_210568055_380000/LConn1 -- T_71500123__Bonaduz/LConn1 -- _CN_71500123_380000_CN156092814/LConn1
  Bonaduz_CN_71500123_380000_CN_210568055_380000/LConn2 -- T_71500123__Bonaduz/LConn2 -- _CN_71500123_380000_CN156092814/LConn2
  Bonaduz_CN_71500123_380000_CN_210568055_380000/LConn3 -- T_71500123__Bonaduz/LConn3 -- _CN_71500123_380000_CN156092814/LConn3 -- bus20/LConn1
  T_210568055__Schaltanlage_Tavanasa/LConn1 -- Bonaduz_CN_71500123_380000_CN_210568055_380000/RConn1
  T_210568055__Schaltanlage_Tavanasa/LConn2 -- Bonaduz_CN_71500123_380000_CN_210568055_380000/RConn2
  Bonaduz_CN_71500123_380000_CN_210568055_380000/RConn3 -- T_210568055__Schaltanlage_Tavanasa/LConn3 -- bus21/LConn1
  T_36348118__Rothenbrunnen/LConn1 -- _CN_71500123_220000_CN_36348118_220000/RConn1
  T_36348118__Rothenbrunnen/LConn2 -- _CN_71500123_220000_CN_36348118_220000/RConn2
  _CN_71500123_220000_CN_36348118_220000/RConn3 -- T_36348118__Rothenbrunnen/LConn3 -- bus22/LConn1
  T_211907009__Unterwerk_Sarelli/LConn1 -- _CN_71500123_220000_CN_211907009_220000/RConn1
  T_211907009__Unterwerk_Sarelli/LConn2 -- _CN_71500123_220000_CN_211907009_220000/RConn2
  _CN_71500123_220000_CN_211907009_220000/RConn3 -- T_211907009__Unterwerk_Sarelli/LConn3 -- bus23/LConn1
  G_156092814_Pumpspeicherkraftwerk_Mapragg/RConn1 -- _CN_71500123_380000_CN156092814/RConn1
  G_156092814_Pumpspeicherkraftwerk_Mapragg/RConn2 -- _CN_71500123_380000_CN156092814/RConn2
  _CN_71500123_380000_CN156092814/RConn3 -- G_156092814_Pumpspeicherkraftwerk_Mapragg/RConn3 -- bus24/LConn1
  _CN_239937062_220000_CN_132373704_220000/LConn1 -- T_239937062__Foretaille/LConn1 -- _CN_239937062_220000_CN_228128829_220000/LConn1 -- _CN_239937062_220000_CN_55698557_220000/LConn1 -- _CN_239937062_220000_CN_55696869_220000/LConn1 -- _CN_239937062_220000_CN_44496892_220000/LConn1
  _CN_239937062_220000_CN_132373704_220000/LConn2 -- T_239937062__Foretaille/LConn2 -- _CN_239937062_220000_CN_228128829_220000/LConn2 -- _CN_239937062_220000_CN_55698557_220000/LConn2 -- _CN_239937062_220000_CN_55696869_220000/LConn2 -- _CN_239937062_220000_CN_44496892_220000/LConn2
  _CN_239937062_220000_CN_132373704_220000/LConn3 -- T_239937062__Foretaille/LConn3 -- _CN_239937062_220000_CN_228128829_220000/LConn3 -- _CN_239937062_220000_CN_55698557_220000/LConn3 -- _CN_239937062_220000_CN_55696869_220000/LConn3 -- bus25/LConn1 -- _CN_239937062_220000_CN_44496892_220000/LConn3
  T_132373704__/LConn1 -- _CN_239937062_220000_CN_132373704_220000/RConn1
  T_132373704__/LConn2 -- _CN_239937062_220000_CN_132373704_220000/RConn2
  _CN_239937062_220000_CN_132373704_220000/RConn3 -- T_132373704__/LConn3 -- bus26/LConn1
  T_44496892__Banlieue_Ouest/LConn1 -- _CN_239937062_220000_CN_44496892_220000/RConn1
  T_44496892__Banlieue_Ouest/LConn2 -- _CN_239937062_220000_CN_44496892_220000/RConn2
  _CN_239937062_220000_CN_44496892_220000/RConn3 -- T_44496892__Banlieue_Ouest/LConn3 -- bus27/LConn1
  T_228128829__/LConn1 -- _CN_239937062_220000_CN_228128829_220000/RConn1
  T_228128829__/LConn2 -- _CN_239937062_220000_CN_228128829_220000/RConn2
  _CN_239937062_220000_CN_228128829_220000/RConn3 -- T_228128829__/LConn3 -- bus28/LConn1
  _CN_239937062_220000_CN_55698557_220000/RConn1 -- T_55698557__St_Triphon/LConn1 -- _CN_55698557_220000_CN_194258388_220000/LConn1
  _CN_239937062_220000_CN_55698557_220000/RConn2 -- T_55698557__St_Triphon/LConn2 -- _CN_55698557_220000_CN_194258388_220000/LConn2
  _CN_239937062_220000_CN_55698557_220000/RConn3 -- T_55698557__St_Triphon/LConn3 -- _CN_55698557_220000_CN_194258388_220000/LConn3 -- bus29/LConn1
  T_55696869__Foretaille/LConn1 -- _CN_239937062_220000_CN_55696869_220000/RConn1
  T_55696869__Foretaille/LConn2 -- _CN_239937062_220000_CN_55696869_220000/RConn2
  _CN_239937062_220000_CN_55696869_220000/RConn3 -- T_55696869__Foretaille/LConn3 -- bus30/LConn1
  T_365590455__Tierfehd/LConn1 -- _CN_192677427_220000_CN_365590455_220000/RConn1
  T_365590455__Tierfehd/LConn2 -- _CN_192677427_220000_CN_365590455_220000/RConn2
  _CN_192677427_220000_CN_365590455_220000/RConn3 -- T_365590455__Tierfehd/LConn3 -- bus31/LConn1
  _CN_89977424_380000_CN_195751829_380000/LConn1 -- T_89977424__/LConn1 -- _CN_89977424_380000_CN_31308888_380000/LConn1
  _CN_89977424_380000_CN_195751829_380000/LConn2 -- T_89977424__/LConn2 -- _CN_89977424_380000_CN_31308888_380000/LConn2
  _CN_89977424_380000_CN_195751829_380000/LConn3 -- T_89977424__/LConn3 -- _CN_89977424_380000_CN_31308888_380000/LConn3 -- bus32/LConn1
  _CN_89977424_380000_CN_195751829_380000/RConn1 -- T_195751829__/LConn1 -- _CN_108257952_380000_CN_195751829_380000/LConn1
  _CN_89977424_380000_CN_195751829_380000/RConn2 -- T_195751829__/LConn2 -- _CN_108257952_380000_CN_195751829_380000/LConn2
  _CN_89977424_380000_CN_195751829_380000/RConn3 -- T_195751829__/LConn3 -- _CN_108257952_380000_CN_195751829_380000/LConn3 -- bus33/LConn1
  T_31308888__Regensdorf/LConn1 -- _CN_89977424_380000_CN_31308888_380000/RConn1
  T_31308888__Regensdorf/LConn2 -- _CN_89977424_380000_CN_31308888_380000/RConn2
  _CN_89977424_380000_CN_31308888_380000/RConn3 -- T_31308888__Regensdorf/LConn3 -- bus34/LConn1
  T_207895647__Ouvras_Electricas_d'Engiadina/LConn1 -- Ova_Spin___Pradella_CN_207895647_220000_CN_26088678_220000/LConn1
  T_207895647__Ouvras_Electricas_d'Engiadina/LConn2 -- Ova_Spin___Pradella_CN_207895647_220000_CN_26088678_220000/LConn2
  Ova_Spin___Pradella_CN_207895647_220000_CN_26088678_220000/LConn3 -- T_207895647__Ouvras_Electricas_d'Engiadina/LConn3 -- bus35/LConn1
  Ova_Spin___Pradella_CN_207895647_220000_CN_26088678_220000/RConn1 -- T_26088678_380000;220000_Pradella/RConn1 -- L_26088678/LConn1
  Ova_Spin___Pradella_CN_207895647_220000_CN_26088678_220000/RConn2 -- T_26088678_380000;220000_Pradella/RConn2 -- L_26088678/LConn2
  Ova_Spin___Pradella_CN_207895647_220000_CN_26088678_220000/RConn3 -- T_26088678_380000;220000_Pradella/RConn3 -- L_26088678/LConn3 -- bus36/LConn1
  T_212498548__/LConn1 -- _CN_212498548_220000_CN212498547/LConn1
  T_212498548__/LConn2 -- _CN_212498548_220000_CN212498547/LConn2
  _CN_212498548_220000_CN212498547/LConn3 -- T_212498548__/LConn3 -- bus37/LConn1
  _CN_212498548_220000_CN212498547/RConn1 -- G_212498547_Kraftwerk_Bärenburg/RConn1 -- _CN_207993342_220000_CN212498547/LConn1
  _CN_212498548_220000_CN212498547/RConn2 -- G_212498547_Kraftwerk_Bärenburg/RConn2 -- _CN_207993342_220000_CN212498547/LConn2
  _CN_212498548_220000_CN212498547/RConn3 -- G_212498547_Kraftwerk_Bärenburg/RConn3 -- _CN_207993342_220000_CN212498547/LConn3 -- bus38/LConn1
  _CN_55698557_220000_CN_194258388_220000/RConn1 -- T_194258388__/LConn1 -- _CN_80266169_220000_CN_194258388_220000/LConn1
  _CN_55698557_220000_CN_194258388_220000/RConn2 -- T_194258388__/LConn2 -- _CN_80266169_220000_CN_194258388_220000/LConn2
  _CN_55698557_220000_CN_194258388_220000/RConn3 -- T_194258388__/LConn3 -- _CN_80266169_220000_CN_194258388_220000/LConn3 -- bus39/LConn1
  T_180138111__/LConn1 -- _CN_180138111_220000_CN_50561341_220000/LConn1
  T_180138111__/LConn2 -- _CN_180138111_220000_CN_50561341_220000/LConn2
  _CN_180138111_220000_CN_50561341_220000/LConn3 -- T_180138111__/LConn3 -- bus40/LConn1
  _CN_180138111_220000_CN_50561341_220000/RConn1 -- T_50561341__/LConn1 -- _CN_180138112_220000_CN_50561341_220000/LConn1 -- _CN_147714395_220000_CN_50561341_220000/RConn1
  _CN_180138111_220000_CN_50561341_220000/RConn2 -- T_50561341__/LConn2 -- _CN_180138112_220000_CN_50561341_220000/LConn2 -- _CN_147714395_220000_CN_50561341_220000/RConn2
  _CN_180138111_220000_CN_50561341_220000/RConn3 -- T_50561341__/LConn3 -- _CN_180138112_220000_CN_50561341_220000/LConn3 -- _CN_147714395_220000_CN_50561341_220000/RConn3 -- bus41/LConn1
  T_180138112__/LConn1 -- _CN_180138112_220000_CN_50561341_220000/RConn1
  T_180138112__/LConn2 -- _CN_180138112_220000_CN_50561341_220000/RConn2
  _CN_180138112_220000_CN_50561341_220000/RConn3 -- T_180138112__/LConn3 -- bus42/LConn1
  _CN_281803398_220000_CN_281812360_220000/LConn1 -- T_281803398__Biasca/LConn1 -- _CN_281803398_220000_CN_281800404_220000/RConn1 -- _CN_281803398_220000_CN_281815404_220000/LConn1
  _CN_281803398_220000_CN_281812360_220000/LConn2 -- T_281803398__Biasca/LConn2 -- _CN_281803398_220000_CN_281800404_220000/RConn2 -- _CN_281803398_220000_CN_281815404_220000/LConn2
  _CN_281803398_220000_CN_281812360_220000/LConn3 -- T_281803398__Biasca/LConn3 -- _CN_281803398_220000_CN_281800404_220000/RConn3 -- _CN_281803398_220000_CN_281815404_220000/LConn3 -- bus43/LConn1
  _CN_281803398_220000_CN_281812360_220000/RConn1 -- T_281812360__/LConn1 -- _CN_281815404_220000_CN_281812360_220000/LConn1
  _CN_281803398_220000_CN_281812360_220000/RConn2 -- T_281812360__/LConn2 -- _CN_281815404_220000_CN_281812360_220000/LConn2
  _CN_281803398_220000_CN_281812360_220000/RConn3 -- T_281812360__/LConn3 -- _CN_281815404_220000_CN_281812360_220000/LConn3 -- bus44/LConn1
  _CN_281803398_220000_CN_281815404_220000/RConn1 -- T_281815404__Magadino/LConn1 -- _CN_281815404_220000_CN_281804158_220000/LConn1 -- _CN_281815404_220000_CN_35487135_220000/LConn1 -- _CN_68186251_220000_CN_281815404_220000/LConn1 -- _CN_281815404_220000_CN_281812360_220000/RConn1
  _CN_281803398_220000_CN_281815404_220000/RConn2 -- T_281815404__Magadino/LConn2 -- _CN_281815404_220000_CN_281804158_220000/LConn2 -- _CN_281815404_220000_CN_35487135_220000/LConn2 -- _CN_68186251_220000_CN_281815404_220000/LConn2 -- _CN_281815404_220000_CN_281812360_220000/RConn2
  _CN_281803398_220000_CN_281815404_220000/RConn3 -- T_281815404__Magadino/LConn3 -- _CN_281815404_220000_CN_281804158_220000/LConn3 -- _CN_281815404_220000_CN_35487135_220000/LConn3 -- bus45/LConn1 -- _CN_68186251_220000_CN_281815404_220000/LConn3 -- _CN_281815404_220000_CN_281812360_220000/RConn3
  _CN_68186251_220000_CN_376534298_220000/LConn1 -- T_68186251__/LConn1 -- _CN_68186251_220000_CN_281815404_220000/RConn1
  _CN_68186251_220000_CN_376534298_220000/LConn2 -- T_68186251__/LConn2 -- _CN_68186251_220000_CN_281815404_220000/RConn2
  _CN_68186251_220000_CN_376534298_220000/LConn3 -- T_68186251__/LConn3 -- _CN_68186251_220000_CN_281815404_220000/RConn3 -- bus46/LConn1
  T_376534298__/LConn1 -- _CN_68186251_220000_CN_376534298_220000/RConn1
  T_376534298__/LConn2 -- _CN_68186251_220000_CN_376534298_220000/RConn2
  _CN_68186251_220000_CN_376534298_220000/RConn3 -- T_376534298__/LConn3 -- bus47/LConn1
  T_97941869__/LConn1 -- _CN_97941869_380000_CN_35002638_380000/LConn1
  T_97941869__/LConn2 -- _CN_97941869_380000_CN_35002638_380000/LConn2
  _CN_97941869_380000_CN_35002638_380000/LConn3 -- T_97941869__/LConn3 -- bus48/LConn1
  _CN_97941869_380000_CN_35002638_380000/RConn1 -- T_35002638__Mettlen/LConn1 -- _CN_40639427_380000_CN_35002638_380000/RConn1 -- _CN_108257952_380000_CN_35002638_380000/LConn1
  _CN_97941869_380000_CN_35002638_380000/RConn2 -- T_35002638__Mettlen/LConn2 -- _CN_40639427_380000_CN_35002638_380000/RConn2 -- _CN_108257952_380000_CN_35002638_380000/LConn2
  _CN_97941869_380000_CN_35002638_380000/RConn3 -- T_35002638__Mettlen/LConn3 -- _CN_40639427_380000_CN_35002638_380000/RConn3 -- _CN_108257952_380000_CN_35002638_380000/LConn3 -- bus49/LConn1
  T_40639427__Gösgen/RConn4 -- _CN_40639427_220000_CN_147557680_220000/LConn1
  T_40639427__Gösgen/RConn5 -- _CN_40639427_220000_CN_147557680_220000/LConn2
  _CN_40639427_220000_CN_147557680_220000/LConn3 -- T_40639427__Gösgen/RConn6 -- bus50/LConn1
  _CN_40639427_220000_CN_147557680_220000/RConn1 -- T_147557680__Unterwerk_Flumenthal/LConn1 -- _CN_147557680_220000_CN_164850030_220000/LConn1
  _CN_40639427_220000_CN_147557680_220000/RConn2 -- T_147557680__Unterwerk_Flumenthal/LConn2 -- _CN_147557680_220000_CN_164850030_220000/LConn2
  _CN_40639427_220000_CN_147557680_220000/RConn3 -- T_147557680__Unterwerk_Flumenthal/LConn3 -- _CN_147557680_220000_CN_164850030_220000/LConn3 -- bus51/LConn1
  T_281810588__Verbano/LConn1 -- Centrale_Verbano___Avegno_CN_281810588_220000_CN_281800404_220000/RConn1
  T_281810588__Verbano/LConn2 -- Centrale_Verbano___Avegno_CN_281810588_220000_CN_281800404_220000/RConn2
  Centrale_Verbano___Avegno_CN_281810588_220000_CN_281800404_220000/RConn3 -- T_281810588__Verbano/LConn3 -- bus52/LConn1
  T_281608861__/LConn1 -- _CN_281608861_220000_CN_228303734_220000/LConn1
  T_281608861__/LConn2 -- _CN_281608861_220000_CN_228303734_220000/LConn2
  _CN_281608861_220000_CN_228303734_220000/LConn3 -- T_281608861__/LConn3 -- bus53/LConn1
  _CN_281608861_220000_CN_228303734_220000/RConn1 -- T_228303734__/LConn1 -- _CN_234983117_220000_CN_228303734_220000/LConn1
  _CN_281608861_220000_CN_228303734_220000/RConn2 -- T_228303734__/LConn2 -- _CN_234983117_220000_CN_228303734_220000/LConn2
  _CN_281608861_220000_CN_228303734_220000/RConn3 -- T_228303734__/LConn3 -- _CN_234983117_220000_CN_228303734_220000/LConn3 -- bus54/LConn1
  _CN_108257952_380000_CN_35002638_380000/RConn1 -- T_108257952__Umspannwerk_Obfelden/LConn1 -- _CN_108257952_380000_CN_195751829_380000/RConn1 -- _CN_108257952_380000_CN_33271433_380000/LConn1
  _CN_108257952_380000_CN_35002638_380000/RConn2 -- T_108257952__Umspannwerk_Obfelden/LConn2 -- _CN_108257952_380000_CN_195751829_380000/RConn2 -- _CN_108257952_380000_CN_33271433_380000/LConn2
  _CN_108257952_380000_CN_35002638_380000/RConn3 -- T_108257952__Umspannwerk_Obfelden/LConn3 -- _CN_108257952_380000_CN_195751829_380000/RConn3 -- _CN_108257952_380000_CN_33271433_380000/LConn3 -- bus55/LConn1
  T_33271433__Niederwil/LConn1 -- _CN_108257952_380000_CN_33271433_380000/RConn1
  T_33271433__Niederwil/LConn2 -- _CN_108257952_380000_CN_33271433_380000/RConn2
  _CN_108257952_380000_CN_33271433_380000/RConn3 -- T_33271433__Niederwil/LConn3 -- bus56/LConn1
  _CN_35840165_380000_CN35840166/LConn1 -- T_35840165_380000_Leibstadt/LConn1 -- _CN_35840165_380000_CN_50319857_380000/RConn1 -- _CN_35840165_380000_CN_98648381_380000/LConn1
  _CN_35840165_380000_CN35840166/LConn2 -- T_35840165_380000_Leibstadt/LConn2 -- _CN_35840165_380000_CN_50319857_380000/RConn2 -- _CN_35840165_380000_CN_98648381_380000/LConn2
  _CN_35840165_380000_CN35840166/LConn3 -- T_35840165_380000_Leibstadt/LConn3 -- _CN_35840165_380000_CN_50319857_380000/RConn3 -- _CN_35840165_380000_CN_98648381_380000/LConn3 -- bus57/LConn1
  G_35840166_Kernkraftwerk_Leibstadt/RConn1 -- _CN_35840165_380000_CN35840166/RConn1
  G_35840166_Kernkraftwerk_Leibstadt/RConn2 -- _CN_35840165_380000_CN35840166/RConn2
  _CN_35840165_380000_CN35840166/RConn3 -- G_35840166_Kernkraftwerk_Leibstadt/RConn3 -- bus58/LConn1
  _CN_35840165_380000_CN_98648381_380000/RConn1 -- T_98648381_380000;220000_Beznau/LConn1 -- _CN_98648381_380000_CN_147714395_380000/LConn1 -- _CN_98648381_380000_CN_50319857_380000/RConn1
  _CN_35840165_380000_CN_98648381_380000/RConn2 -- T_98648381_380000;220000_Beznau/LConn2 -- _CN_98648381_380000_CN_147714395_380000/LConn2 -- _CN_98648381_380000_CN_50319857_380000/RConn2
  _CN_35840165_380000_CN_98648381_380000/RConn3 -- T_98648381_380000;220000_Beznau/LConn3 -- _CN_98648381_380000_CN_147714395_380000/LConn3 -- bus59/LConn1 -- _CN_98648381_380000_CN_50319857_380000/RConn3
  _CN_402055336_220000_CN_234983117_220000/LConn1 -- T_402055336__Gstaad/LConn1 -- _CN_402055336_220000_CN_384104425_220000/LConn1
  _CN_402055336_220000_CN_234983117_220000/LConn2 -- T_402055336__Gstaad/LConn2 -- _CN_402055336_220000_CN_384104425_220000/LConn2
  _CN_402055336_220000_CN_234983117_220000/LConn3 -- T_402055336__Gstaad/LConn3 -- _CN_402055336_220000_CN_384104425_220000/LConn3 -- bus60/LConn1
  _CN_402055336_220000_CN_234983117_220000/RConn1 -- T_234983117__Chamoson/LConn1 -- _CN_234983117_220000_CN_212722603_220000/LConn1 -- _CN_234983117_220000_CN_228303734_220000/RConn1
  _CN_402055336_220000_CN_234983117_220000/RConn2 -- T_234983117__Chamoson/LConn2 -- _CN_234983117_220000_CN_212722603_220000/LConn2 -- _CN_234983117_220000_CN_228303734_220000/RConn2
  _CN_402055336_220000_CN_234983117_220000/RConn3 -- T_234983117__Chamoson/LConn3 -- _CN_234983117_220000_CN_212722603_220000/LConn3 -- _CN_234983117_220000_CN_228303734_220000/RConn3 -- bus61/LConn1
  _CN_402055336_220000_CN_384104425_220000/RConn1 -- T_384104425__/LConn1 -- _CN_34238394_220000_CN_384104425_220000/LConn1
  _CN_402055336_220000_CN_384104425_220000/RConn2 -- T_384104425__/LConn2 -- _CN_34238394_220000_CN_384104425_220000/LConn2
  _CN_402055336_220000_CN_384104425_220000/RConn3 -- T_384104425__/LConn3 -- _CN_34238394_220000_CN_384104425_220000/LConn3 -- bus62/LConn1
  T_165513396__/LConn1 -- _CN_165513396_220000_CN_89405664_220000/LConn1
  T_165513396__/LConn2 -- _CN_165513396_220000_CN_89405664_220000/LConn2
  _CN_165513396_220000_CN_89405664_220000/LConn3 -- T_165513396__/LConn3 -- bus63/LConn1
  _CN_165513396_220000_CN_89405664_220000/RConn1 -- T_89405664_220000;132000;15000_Rupperswil/LConn1 -- _CN_89405664_220000_CN_190819048_220000/LConn1
  _CN_165513396_220000_CN_89405664_220000/RConn2 -- T_89405664_220000;132000;15000_Rupperswil/LConn2 -- _CN_89405664_220000_CN_190819048_220000/LConn2
  _CN_165513396_220000_CN_89405664_220000/RConn3 -- T_89405664_220000;132000;15000_Rupperswil/LConn3 -- _CN_89405664_220000_CN_190819048_220000/LConn3 -- bus64/LConn1
  T_83861269_220000_Montlingen/LConn1 -- Stoss_Süd;Falknis_CN_92798668_220000_CN_83861269_220000/RConn1
  T_83861269_220000_Montlingen/LConn2 -- Stoss_Süd;Falknis_CN_92798668_220000_CN_83861269_220000/RConn2
  Stoss_Süd;Falknis_CN_92798668_220000_CN_83861269_220000/RConn3 -- T_83861269_220000_Montlingen/LConn3 -- bus65/LConn1
  T_92873516_220000_Mörschwil/LConn1 -- Stoss_Süd;Falknis_CN_92798668_220000_CN_92873516_220000/RConn1
  T_92873516_220000_Mörschwil/LConn2 -- Stoss_Süd;Falknis_CN_92798668_220000_CN_92873516_220000/RConn2
  Stoss_Süd;Falknis_CN_92798668_220000_CN_92873516_220000/RConn3 -- T_92873516_220000_Mörschwil/LConn3 -- bus66/LConn1
  T_212722603__/LConn1 -- _CN_234983117_220000_CN_212722603_220000/RConn1
  T_212722603__/LConn2 -- _CN_234983117_220000_CN_212722603_220000/RConn2
  _CN_234983117_220000_CN_212722603_220000/RConn3 -- T_212722603__/LConn3 -- bus67/LConn1
  T_197031131__/LConn1 -- _CN_197031131_220000_CN_127004407_220000/LConn1
  T_197031131__/LConn2 -- _CN_197031131_220000_CN_127004407_220000/LConn2
  _CN_197031131_220000_CN_127004407_220000/LConn3 -- T_197031131__/LConn3 -- bus68/LConn1
  _CN_197031131_220000_CN_127004407_220000/RConn1 -- T_127004407_380000;220000_Bassecourt/RConn1 -- L_127004407/LConn1
  _CN_197031131_220000_CN_127004407_220000/RConn2 -- T_127004407_380000;220000_Bassecourt/RConn2 -- L_127004407/LConn2
  _CN_197031131_220000_CN_127004407_220000/RConn3 -- T_127004407_380000;220000_Bassecourt/RConn3 -- L_127004407/LConn3 -- bus69/LConn1
  _CN_89405664_220000_CN_190819048_220000/RConn1 -- T_190819048__Oftringen/LConn1 -- _CN_190819048_220000_CN_402053379_220000/LConn1 -- _CN_190819048_220000_CN_164850030_220000/LConn1 -- _CN_190819048_220000_CN_50319857_220000/LConn1
  _CN_89405664_220000_CN_190819048_220000/RConn2 -- T_190819048__Oftringen/LConn2 -- _CN_190819048_220000_CN_402053379_220000/LConn2 -- _CN_190819048_220000_CN_164850030_220000/LConn2 -- _CN_190819048_220000_CN_50319857_220000/LConn2
  _CN_89405664_220000_CN_190819048_220000/RConn3 -- T_190819048__Oftringen/LConn3 -- _CN_190819048_220000_CN_402053379_220000/LConn3 -- _CN_190819048_220000_CN_164850030_220000/LConn3 -- _CN_190819048_220000_CN_50319857_220000/LConn3 -- bus70/LConn1
  _CN_26088678_380000_CN_207993342_380000/LConn1 -- T_26088678_380000;220000_Pradella/LConn1 -- _CN_26088678_380000_CN_207991759_380000/LConn1
  _CN_26088678_380000_CN_207993342_380000/LConn2 -- T_26088678_380000;220000_Pradella/LConn2 -- _CN_26088678_380000_CN_207991759_380000/LConn2
  _CN_26088678_380000_CN_207993342_380000/LConn3 -- T_26088678_380000;220000_Pradella/LConn3 -- _CN_26088678_380000_CN_207991759_380000/LConn3 -- bus71/LConn1
  _CN_26088678_380000_CN_207993342_380000/RConn1 -- T_207993342_380000;220000_Schaltanlage_Sils_i__D_/LConn1 -- _CN_193131937_380000_CN_207993342_380000/LConn1
  _CN_26088678_380000_CN_207993342_380000/RConn2 -- T_207993342_380000;220000_Schaltanlage_Sils_i__D_/LConn2 -- _CN_193131937_380000_CN_207993342_380000/LConn2
  _CN_26088678_380000_CN_207993342_380000/RConn3 -- T_207993342_380000;220000_Schaltanlage_Sils_i__D_/LConn3 -- _CN_193131937_380000_CN_207993342_380000/LConn3 -- bus72/LConn1
  T_207991759_380000_Robbia/LConn1 -- _CN_26088678_380000_CN_207991759_380000/RConn1
  T_207991759_380000_Robbia/LConn2 -- _CN_26088678_380000_CN_207991759_380000/RConn2
  _CN_26088678_380000_CN_207991759_380000/RConn3 -- T_207991759_380000_Robbia/LConn3 -- bus73/LConn1
  T_402053379_220000_Lindenholz/LConn1 -- _CN_190819048_220000_CN_402053379_220000/RConn1
  T_402053379_220000_Lindenholz/LConn2 -- _CN_190819048_220000_CN_402053379_220000/RConn2
  _CN_190819048_220000_CN_402053379_220000/RConn3 -- T_402053379_220000_Lindenholz/LConn3 -- bus74/LConn1
  _CN_190819048_220000_CN_164850030_220000/RConn1 -- T_164850030__Bickingen/LConn1 -- _CN_35002638_220000_CN_164850030_220000/RConn1 -- _CN_147557680_220000_CN_164850030_220000/RConn1
  _CN_190819048_220000_CN_164850030_220000/RConn2 -- T_164850030__Bickingen/LConn2 -- _CN_35002638_220000_CN_164850030_220000/RConn2 -- _CN_147557680_220000_CN_164850030_220000/RConn2
  _CN_190819048_220000_CN_164850030_220000/RConn3 -- T_164850030__Bickingen/LConn3 -- _CN_35002638_220000_CN_164850030_220000/RConn3 -- _CN_147557680_220000_CN_164850030_220000/RConn3 -- bus75/LConn1
  _CN_190819048_220000_CN_50319857_220000/RConn1 -- T_50319857_380000;220000_Laufenburg/RConn1 -- _CN_98648381_220000_CN_50319857_220000/LConn1 -- L_50319857/LConn1 -- _CN_109037817_220000_CN_50319857_220000/LConn1
  _CN_190819048_220000_CN_50319857_220000/RConn2 -- T_50319857_380000;220000_Laufenburg/RConn2 -- _CN_98648381_220000_CN_50319857_220000/LConn2 -- L_50319857/LConn2 -- _CN_109037817_220000_CN_50319857_220000/LConn2
  _CN_190819048_220000_CN_50319857_220000/RConn3 -- T_50319857_380000;220000_Laufenburg/RConn3 -- _CN_98648381_220000_CN_50319857_220000/LConn3 -- L_50319857/LConn3 -- bus76/LConn1 -- _CN_109037817_220000_CN_50319857_220000/LConn3
  T_236819191__/LConn1 -- _CN_236819191_220000_CN_228003081_220000/LConn1
  T_236819191__/LConn2 -- _CN_236819191_220000_CN_228003081_220000/LConn2
  _CN_236819191_220000_CN_228003081_220000/LConn3 -- T_236819191__/LConn3 -- bus77/LConn1
  T_228003081__/LConn1 -- _CN_236819191_220000_CN_228003081_220000/RConn1
  T_228003081__/LConn2 -- _CN_236819191_220000_CN_228003081_220000/RConn2
  _CN_236819191_220000_CN_228003081_220000/RConn3 -- T_228003081__/LConn3 -- bus78/LConn1
  _CN_109037817_220000_CN_50319857_220000/RConn1 -- T_109037817_220000_Lachmatt/LConn1 -- _CN_109037817_220000_CN_109029720_220000/LConn1
  _CN_109037817_220000_CN_50319857_220000/RConn2 -- T_109037817_220000_Lachmatt/LConn2 -- _CN_109037817_220000_CN_109029720_220000/LConn2
  _CN_109037817_220000_CN_50319857_220000/RConn3 -- T_109037817_220000_Lachmatt/LConn3 -- _CN_109037817_220000_CN_109029720_220000/LConn3 -- bus79/LConn1
  T_109029720__Münchwilen/LConn1 -- _CN_109037817_220000_CN_109029720_220000/RConn1
  T_109029720__Münchwilen/LConn2 -- _CN_109037817_220000_CN_109029720_220000/RConn2
  _CN_109037817_220000_CN_109029720_220000/RConn3 -- T_109029720__Münchwilen/LConn3 -- bus80/LConn1
  _CN_397960460_380000_CN_30350721_380000/LConn1 -- T_397960460_380000_Asphard/LConn1 -- _CN_397960460_380000_CN_50319857_380000/RConn1
  _CN_397960460_380000_CN_30350721_380000/LConn2 -- T_397960460_380000_Asphard/LConn2 -- _CN_397960460_380000_CN_50319857_380000/RConn2
  _CN_397960460_380000_CN_30350721_380000/LConn3 -- T_397960460_380000_Asphard/LConn3 -- _CN_397960460_380000_CN_50319857_380000/RConn3 -- bus81/LConn1
  T_30350721__Ormalingen/LConn1 -- _CN_397960460_380000_CN_30350721_380000/RConn1
  T_30350721__Ormalingen/LConn2 -- _CN_397960460_380000_CN_30350721_380000/RConn2
  _CN_397960460_380000_CN_30350721_380000/RConn3 -- T_30350721__Ormalingen/LConn3 -- bus82/LConn1
  T_240959264__/LConn1 -- _CN_240959264_220000_CN_26166640_220000/LConn1
  T_240959264__/LConn2 -- _CN_240959264_220000_CN_26166640_220000/LConn2
  _CN_240959264_220000_CN_26166640_220000/LConn3 -- T_240959264__/LConn3 -- bus83/LConn1
  T_26166640_220000_Unterstation_Wattenwil_(BKW_Energie)/LConn1 -- _CN_240959264_220000_CN_26166640_220000/RConn1
  T_26166640_220000_Unterstation_Wattenwil_(BKW_Energie)/LConn2 -- _CN_240959264_220000_CN_26166640_220000/RConn2
  _CN_240959264_220000_CN_26166640_220000/RConn3 -- T_26166640_220000_Unterstation_Wattenwil_(BKW_Energie)/LConn3 -- bus84/LConn1
  T_161853746__/LConn1 -- _CN_161853746_220000_CN_80266169_220000/LConn1
  T_161853746__/LConn2 -- _CN_161853746_220000_CN_80266169_220000/LConn2
  _CN_161853746_220000_CN_80266169_220000/LConn3 -- T_161853746__/LConn3 -- bus85/LConn1
  _CN_161853746_220000_CN_80266169_220000/RConn1 -- T_80266169__Mühleberg_West/LConn1 -- _CN_80266169_220000_CN_34238394_220000/LConn1 -- _CN_80266169_220000_CN_163881972_220000/LConn1 -- _CN_80266169_220000_CN_194258388_220000/RConn1
  _CN_161853746_220000_CN_80266169_220000/RConn2 -- T_80266169__Mühleberg_West/LConn2 -- _CN_80266169_220000_CN_34238394_220000/LConn2 -- _CN_80266169_220000_CN_163881972_220000/LConn2 -- _CN_80266169_220000_CN_194258388_220000/RConn2
  _CN_161853746_220000_CN_80266169_220000/RConn3 -- T_80266169__Mühleberg_West/LConn3 -- _CN_80266169_220000_CN_34238394_220000/LConn3 -- _CN_80266169_220000_CN_163881972_220000/LConn3 -- bus86/LConn1 -- _CN_80266169_220000_CN_194258388_220000/RConn3
  T_100662075__Sedrun/LConn1 -- _CN_100662075_220000_CN_210568055_220000/RConn1
  T_100662075__Sedrun/LConn2 -- _CN_100662075_220000_CN_210568055_220000/RConn2
  _CN_100662075_220000_CN_210568055_220000/RConn3 -- T_100662075__Sedrun/LConn3 -- bus87/LConn1
  _CN_98648381_220000_CN_27107779_220000/LConn1 -- T_98648381_380000;220000_Beznau/RConn1 -- _CN_98648381_220000_CN_50319857_220000/RConn1 -- L_98648381/LConn1
  _CN_98648381_220000_CN_27107779_220000/LConn2 -- T_98648381_380000;220000_Beznau/RConn2 -- _CN_98648381_220000_CN_50319857_220000/RConn2 -- L_98648381/LConn2
  _CN_98648381_220000_CN_27107779_220000/LConn3 -- T_98648381_380000;220000_Beznau/RConn3 -- _CN_98648381_220000_CN_50319857_220000/RConn3 -- L_98648381/LConn3 -- bus88/LConn1
  T_27107779_220000_Eglisau/LConn1 -- _CN_98648381_220000_CN_27107779_220000/RConn1
  T_27107779_220000_Eglisau/LConn2 -- _CN_98648381_220000_CN_27107779_220000/RConn2
  _CN_98648381_220000_CN_27107779_220000/RConn3 -- T_27107779_220000_Eglisau/LConn3 -- bus89/LConn1
  T_147714395__/LConn1 -- _CN_98648381_380000_CN_147714395_380000/RConn1
  T_147714395__/LConn2 -- _CN_98648381_380000_CN_147714395_380000/RConn2
  _CN_98648381_380000_CN_147714395_380000/RConn3 -- T_147714395__/LConn3 -- bus90/LConn1
  _CN_329659200_220000_CN75243304/LConn1 -- T_329659200__Lastverteilerwerk_Neubrück/LConn1 -- _CN_329659200_220000_CN_34238394_220000/LConn1
  _CN_329659200_220000_CN75243304/LConn2 -- T_329659200__Lastverteilerwerk_Neubrück/LConn2 -- _CN_329659200_220000_CN_34238394_220000/LConn2
  _CN_329659200_220000_CN75243304/LConn3 -- T_329659200__Lastverteilerwerk_Neubrück/LConn3 -- _CN_329659200_220000_CN_34238394_220000/LConn3 -- bus91/LConn1
  G_75243304_/RConn1 -- _CN_329659200_220000_CN75243304/RConn1
  G_75243304_/RConn2 -- _CN_329659200_220000_CN75243304/RConn2
  _CN_329659200_220000_CN75243304/RConn3 -- G_75243304_/RConn3 -- bus92/LConn1
  _CN_329659200_220000_CN_34238394_220000/RConn1 -- T_34238394_220000_Mühleberg_Ost/LConn1 -- _CN_80266169_220000_CN_34238394_220000/RConn1 -- _CN_34238394_220000_CN_384104425_220000/RConn1
  _CN_329659200_220000_CN_34238394_220000/RConn2 -- T_34238394_220000_Mühleberg_Ost/LConn2 -- _CN_80266169_220000_CN_34238394_220000/RConn2 -- _CN_34238394_220000_CN_384104425_220000/RConn2
  _CN_329659200_220000_CN_34238394_220000/RConn3 -- T_34238394_220000_Mühleberg_Ost/LConn3 -- _CN_80266169_220000_CN_34238394_220000/RConn3 -- _CN_34238394_220000_CN_384104425_220000/RConn3 -- bus93/LConn1
  T_87281514__/LConn1 -- _CN_147714395_220000_CN_87281514_220000/RConn1
  T_87281514__/LConn2 -- _CN_147714395_220000_CN_87281514_220000/RConn2
  _CN_147714395_220000_CN_87281514_220000/RConn3 -- T_87281514__/LConn3 -- bus94/LConn1
  T_208623457__/LConn1 -- _CN_208623457_220000_CN107244422/LConn1
  T_208623457__/LConn2 -- _CN_208623457_220000_CN107244422/LConn2
  _CN_208623457_220000_CN107244422/LConn3 -- T_208623457__/LConn3 -- bus95/LConn1
  G_107244422_ewz_Tinizong/RConn1 -- _CN_208623457_220000_CN107244422/RConn1
  G_107244422_ewz_Tinizong/RConn2 -- _CN_208623457_220000_CN107244422/RConn2
  _CN_208623457_220000_CN107244422/RConn3 -- G_107244422_ewz_Tinizong/RConn3 -- bus96/LConn1
  T_196539748__/LConn1 -- _CN_196539748_380000_CN_127004407_380000/LConn1
  T_196539748__/LConn2 -- _CN_196539748_380000_CN_127004407_380000/LConn2
  _CN_196539748_380000_CN_127004407_380000/LConn3 -- T_196539748__/LConn3 -- bus97/LConn1
  _CN_196539748_380000_CN_127004407_380000/RConn1 -- T_127004407_380000;220000_Bassecourt/LConn1 -- _CN_164850027_380000_CN_127004407_380000/LConn1
  _CN_196539748_380000_CN_127004407_380000/RConn2 -- T_127004407_380000;220000_Bassecourt/LConn2 -- _CN_164850027_380000_CN_127004407_380000/LConn2
  _CN_196539748_380000_CN_127004407_380000/RConn3 -- T_127004407_380000;220000_Bassecourt/LConn3 -- _CN_164850027_380000_CN_127004407_380000/LConn3 -- bus98/LConn1
  _CN_164850027_380000_CN_127004407_380000/RConn1 -- T_164850027__Bickigen/LConn1 -- _CN_164850027_380000_CN_50319857_380000/RConn1
  _CN_164850027_380000_CN_127004407_380000/RConn2 -- T_164850027__Bickigen/LConn2 -- _CN_164850027_380000_CN_50319857_380000/RConn2
  _CN_164850027_380000_CN_127004407_380000/RConn3 -- T_164850027__Bickigen/LConn3 -- _CN_164850027_380000_CN_50319857_380000/RConn3 -- bus99/LConn1
  T_281804158__Soazza/LConn1 -- _CN_281815404_220000_CN_281804158_220000/RConn1
  T_281804158__Soazza/LConn2 -- _CN_281815404_220000_CN_281804158_220000/RConn2
  _CN_281815404_220000_CN_281804158_220000/RConn3 -- T_281804158__Soazza/LConn3 -- bus100/LConn1
  T_35487135__/LConn1 -- _CN_281815404_220000_CN_35487135_220000/RConn1
  T_35487135__/LConn2 -- _CN_281815404_220000_CN_35487135_220000/RConn2
  _CN_281815404_220000_CN_35487135_220000/RConn3 -- T_35487135__/LConn3 -- bus101/LConn1
  T_57038202__/LConn1 -- Ligne_220_kV_en_souterrain_CN_57038202_220000_CN_57038204_220000/LConn1
  T_57038202__/LConn2 -- Ligne_220_kV_en_souterrain_CN_57038202_220000_CN_57038204_220000/LConn2
  Ligne_220_kV_en_souterrain_CN_57038202_220000_CN_57038204_220000/LConn3 -- T_57038202__/LConn3 -- bus102/LConn1
  T_57038204__/LConn1 -- Ligne_220_kV_en_souterrain_CN_57038202_220000_CN_57038204_220000/RConn1
  T_57038204__/LConn2 -- Ligne_220_kV_en_souterrain_CN_57038202_220000_CN_57038204_220000/RConn2
  Ligne_220_kV_en_souterrain_CN_57038202_220000_CN_57038204_220000/RConn3 -- T_57038204__/LConn3 -- bus103/LConn1
  T_27435934_220000_Froloo/LConn1 -- _CN_30350721_220000_CN_27435934_220000/RConn1
  T_27435934_220000_Froloo/LConn2 -- _CN_30350721_220000_CN_27435934_220000/RConn2
  _CN_30350721_220000_CN_27435934_220000/RConn3 -- T_27435934_220000_Froloo/LConn3 -- bus104/LConn1
  _CN_11282314_220000_CN_193131937_220000/RConn1 -- T_193131937__/RConn1 -- _CN_193131937_220000_CN_207993342_220000/LConn1
  _CN_11282314_220000_CN_193131937_220000/RConn2 -- T_193131937__/RConn2 -- _CN_193131937_220000_CN_207993342_220000/LConn2
  _CN_11282314_220000_CN_193131937_220000/RConn3 -- T_193131937__/RConn3 -- _CN_193131937_220000_CN_207993342_220000/LConn3 -- bus105/LConn1
  T_193131937__/LConn1 -- _CN_193131937_380000_CN_207993342_380000/RConn1
  T_193131937__/LConn2 -- _CN_193131937_380000_CN_207993342_380000/RConn2
  _CN_193131937_380000_CN_207993342_380000/RConn3 -- T_193131937__/LConn3 -- bus106/LConn1
  _CN_193131937_220000_CN_207993342_220000/RConn1 -- T_207993342_380000;220000_Schaltanlage_Sils_i__D_/RConn1 -- _CN_207993342_220000_CN212498547/RConn1 -- L_207993342/LConn1
  _CN_193131937_220000_CN_207993342_220000/RConn2 -- T_207993342_380000;220000_Schaltanlage_Sils_i__D_/RConn2 -- _CN_207993342_220000_CN212498547/RConn2 -- L_207993342/LConn2
  _CN_193131937_220000_CN_207993342_220000/RConn3 -- T_207993342_380000;220000_Schaltanlage_Sils_i__D_/RConn3 -- _CN_207993342_220000_CN212498547/RConn3 -- L_207993342/LConn3 -- bus107/LConn1
  T_163881972__/LConn1 -- _CN_80266169_220000_CN_163881972_220000/RConn1
  T_163881972__/LConn2 -- _CN_80266169_220000_CN_163881972_220000/RConn2
  _CN_80266169_220000_CN_163881972_220000/RConn3 -- T_163881972__/LConn3 -- bus108/LConn1
  T_140873735__/RConn1 -- L_140873735/LConn1
  T_140873735__/RConn2 -- L_140873735/LConn2
  L_140873735/LConn3 -- T_140873735__/RConn3 -- bus109/LConn1
  T_281800404__Umspannwerk_Avegno/RConn1 -- L_281800404/LConn1
  T_281800404__Umspannwerk_Avegno/RConn2 -- L_281800404/LConn2
  L_281800404/LConn3 -- T_281800404__Umspannwerk_Avegno/RConn3 -- bus110/LConn1
  T_356292116__/RConn1 -- L_356292116/LConn1
  T_356292116__/RConn2 -- L_356292116/LConn2
  L_356292116/LConn3 -- T_356292116__/RConn3 -- bus111/LConn1
  T_40639427__Gösgen/RConn1 -- L_40639427/LConn1
  T_40639427__Gösgen/RConn2 -- L_40639427/LConn2
  L_40639427/LConn3 -- T_40639427__Gösgen/RConn3 -- bus112/LConn1
  T_30350721__Ormalingen/RConn4 -- L_30350721/LConn1
  T_30350721__Ormalingen/RConn5 -- L_30350721/LConn2
  L_30350721/LConn3 -- T_30350721__Ormalingen/RConn6 -- bus113/LConn1
  T_146225999__Sursee/RConn1 -- L_146225999/LConn1
  T_146225999__Sursee/RConn2 -- L_146225999/LConn2
  L_146225999/LConn3 -- T_146225999__Sursee/RConn3 -- bus114/LConn1
  T_35002638__Mettlen/RConn4 -- L_35002638/LConn1
  T_35002638__Mettlen/RConn5 -- L_35002638/LConn2
  L_35002638/LConn3 -- T_35002638__Mettlen/RConn6 -- bus115/LConn1
  T_26843160_220000_Weinfelden/RConn1 -- L_26843160/LConn1
  T_26843160_220000_Weinfelden/RConn2 -- L_26843160/LConn2
  L_26843160/LConn3 -- T_26843160_220000_Weinfelden/RConn3 -- bus116/LConn1
  T_147714395__/RConn4 -- L_147714395/LConn1
  T_147714395__/RConn5 -- L_147714395/LConn2
  L_147714395/LConn3 -- T_147714395__/RConn6 -- bus117/LConn1
  T_240575085_220000_Aathal/RConn1 -- L_240575085/LConn1
  T_240575085_220000_Aathal/RConn2 -- L_240575085/LConn2
  L_240575085/LConn3 -- T_240575085_220000_Aathal/RConn3 -- bus118/LConn1
  T_192677427_380000;220000_Grynau/RConn1 -- L_192677427/LConn1
  T_192677427_380000;220000_Grynau/RConn2 -- L_192677427/LConn2
  L_192677427/LConn3 -- T_192677427_380000;220000_Grynau/RConn3 -- bus119/LConn1
  T_11282314__Unterwerk_Fällanden/RConn1 -- L_11282314/LConn1
  T_11282314__Unterwerk_Fällanden/RConn2 -- L_11282314/LConn2
  L_11282314/LConn3 -- T_11282314__Unterwerk_Fällanden/RConn3 -- bus120/LConn1
  T_92798668_220000_Winkeln/RConn1 -- L_92798668/LConn1
  T_92798668_220000_Winkeln/RConn2 -- L_92798668/LConn2
  L_92798668/LConn3 -- T_92798668_220000_Winkeln/RConn3 -- bus121/LConn1
  T_71500123__Bonaduz/RConn4 -- L_71500123/LConn1
  T_71500123__Bonaduz/RConn5 -- L_71500123/LConn2
  L_71500123/LConn3 -- T_71500123__Bonaduz/RConn6 -- bus122/LConn1
  T_365556107__Ilanz/RConn1 -- L_365556107/LConn1
  T_365556107__Ilanz/RConn2 -- L_365556107/LConn2
  L_365556107/LConn3 -- T_365556107__Ilanz/RConn3 -- bus123/LConn1
  T_210568055__Schaltanlage_Tavanasa/RConn4 -- L_210568055/LConn1
  T_210568055__Schaltanlage_Tavanasa/RConn5 -- L_210568055/LConn2
  L_210568055/LConn3 -- T_210568055__Schaltanlage_Tavanasa/RConn6 -- bus124/LConn1
  T_36348118__Rothenbrunnen/RConn1 -- L_36348118/LConn1
  T_36348118__Rothenbrunnen/RConn2 -- L_36348118/LConn2
  L_36348118/LConn3 -- T_36348118__Rothenbrunnen/RConn3 -- bus125/LConn1
  T_211907009__Unterwerk_Sarelli/RConn1 -- L_211907009/LConn1
  T_211907009__Unterwerk_Sarelli/RConn2 -- L_211907009/LConn2
  L_211907009/LConn3 -- T_211907009__Unterwerk_Sarelli/RConn3 -- bus126/LConn1
  T_239937062__Foretaille/RConn1 -- L_239937062/LConn1
  T_239937062__Foretaille/RConn2 -- L_239937062/LConn2
  L_239937062/LConn3 -- T_239937062__Foretaille/RConn3 -- bus127/LConn1
  T_132373704__/RConn1 -- L_132373704/LConn1
  T_132373704__/RConn2 -- L_132373704/LConn2
  L_132373704/LConn3 -- T_132373704__/RConn3 -- bus128/LConn1
  T_44496892__Banlieue_Ouest/RConn1 -- L_44496892/LConn1
  T_44496892__Banlieue_Ouest/RConn2 -- L_44496892/LConn2
  L_44496892/LConn3 -- T_44496892__Banlieue_Ouest/RConn3 -- bus129/LConn1
  T_228128829__/RConn1 -- L_228128829/LConn1
  T_228128829__/RConn2 -- L_228128829/LConn2
  L_228128829/LConn3 -- T_228128829__/RConn3 -- bus130/LConn1
  T_55698557__St_Triphon/RConn1 -- L_55698557/LConn1
  T_55698557__St_Triphon/RConn2 -- L_55698557/LConn2
  L_55698557/LConn3 -- T_55698557__St_Triphon/RConn3 -- bus131/LConn1
  T_55696869__Foretaille/RConn1 -- L_55696869/LConn1
  T_55696869__Foretaille/RConn2 -- L_55696869/LConn2
  L_55696869/LConn3 -- T_55696869__Foretaille/RConn3 -- bus132/LConn1
  T_365590455__Tierfehd/RConn1 -- L_365590455/LConn1
  T_365590455__Tierfehd/RConn2 -- L_365590455/LConn2
  L_365590455/LConn3 -- T_365590455__Tierfehd/RConn3 -- bus133/LConn1
  T_89977424__/RConn1 -- L_89977424/LConn1
  T_89977424__/RConn2 -- L_89977424/LConn2
  L_89977424/LConn3 -- T_89977424__/RConn3 -- bus134/LConn1
  T_195751829__/RConn1 -- L_195751829/LConn1
  T_195751829__/RConn2 -- L_195751829/LConn2
  L_195751829/LConn3 -- T_195751829__/RConn3 -- bus135/LConn1
  T_31308888__Regensdorf/RConn1 -- L_31308888/LConn1
  T_31308888__Regensdorf/RConn2 -- L_31308888/LConn2
  L_31308888/LConn3 -- T_31308888__Regensdorf/RConn3 -- bus136/LConn1
  T_207895647__Ouvras_Electricas_d'Engiadina/RConn1 -- L_207895647/LConn1
  T_207895647__Ouvras_Electricas_d'Engiadina/RConn2 -- L_207895647/LConn2
  L_207895647/LConn3 -- T_207895647__Ouvras_Electricas_d'Engiadina/RConn3 -- bus137/LConn1
  T_212498548__/RConn1 -- L_212498548/LConn1
  T_212498548__/RConn2 -- L_212498548/LConn2
  L_212498548/LConn3 -- T_212498548__/RConn3 -- bus138/LConn1
  T_194258388__/RConn1 -- L_194258388/LConn1
  T_194258388__/RConn2 -- L_194258388/LConn2
  L_194258388/LConn3 -- T_194258388__/RConn3 -- bus139/LConn1
  T_180138111__/RConn1 -- L_180138111/LConn1
  T_180138111__/RConn2 -- L_180138111/LConn2
  L_180138111/LConn3 -- T_180138111__/RConn3 -- bus140/LConn1
  T_50561341__/RConn1 -- L_50561341/LConn1
  T_50561341__/RConn2 -- L_50561341/LConn2
  L_50561341/LConn3 -- T_50561341__/RConn3 -- bus141/LConn1
  T_180138112__/RConn1 -- L_180138112/LConn1
  T_180138112__/RConn2 -- L_180138112/LConn2
  L_180138112/LConn3 -- T_180138112__/RConn3 -- bus142/LConn1
  T_281803398__Biasca/RConn1 -- L_281803398/LConn1
  T_281803398__Biasca/RConn2 -- L_281803398/LConn2
  L_281803398/LConn3 -- T_281803398__Biasca/RConn3 -- bus143/LConn1
  T_281812360__/RConn1 -- L_281812360/LConn1
  T_281812360__/RConn2 -- L_281812360/LConn2
  L_281812360/LConn3 -- T_281812360__/RConn3 -- bus144/LConn1
  T_281815404__Magadino/RConn1 -- L_281815404/LConn1
  T_281815404__Magadino/RConn2 -- L_281815404/LConn2
  L_281815404/LConn3 -- T_281815404__Magadino/RConn3 -- bus145/LConn1
  T_68186251__/RConn1 -- L_68186251/LConn1
  T_68186251__/RConn2 -- L_68186251/LConn2
  L_68186251/LConn3 -- T_68186251__/RConn3 -- bus146/LConn1
  T_376534298__/RConn1 -- L_376534298/LConn1
  T_376534298__/RConn2 -- L_376534298/LConn2
  L_376534298/LConn3 -- T_376534298__/RConn3 -- bus147/LConn1
  T_97941869__/RConn1 -- L_97941869/LConn1
  T_97941869__/RConn2 -- L_97941869/LConn2
  L_97941869/LConn3 -- T_97941869__/RConn3 -- bus148/LConn1
  T_147557680__Unterwerk_Flumenthal/RConn1 -- L_147557680/LConn1
  T_147557680__Unterwerk_Flumenthal/RConn2 -- L_147557680/LConn2
  L_147557680/LConn3 -- T_147557680__Unterwerk_Flumenthal/RConn3 -- bus149/LConn1
  T_281810588__Verbano/RConn1 -- L_281810588/LConn1
  T_281810588__Verbano/RConn2 -- L_281810588/LConn2
  L_281810588/LConn3 -- T_281810588__Verbano/RConn3 -- bus150/LConn1
  T_281608861__/RConn1 -- L_281608861/LConn1
  T_281608861__/RConn2 -- L_281608861/LConn2
  L_281608861/LConn3 -- T_281608861__/RConn3 -- bus151/LConn1
  T_228303734__/RConn1 -- L_228303734/LConn1
  T_228303734__/RConn2 -- L_228303734/LConn2
  L_228303734/LConn3 -- T_228303734__/RConn3 -- bus152/LConn1
  T_108257952__Umspannwerk_Obfelden/RConn1 -- L_108257952/LConn1
  T_108257952__Umspannwerk_Obfelden/RConn2 -- L_108257952/LConn2
  L_108257952/LConn3 -- T_108257952__Umspannwerk_Obfelden/RConn3 -- bus153/LConn1
  T_33271433__Niederwil/RConn1 -- L_33271433/LConn1
  T_33271433__Niederwil/RConn2 -- L_33271433/LConn2
  L_33271433/LConn3 -- T_33271433__Niederwil/RConn3 -- bus154/LConn1
  T_35840165_380000_Leibstadt/RConn1 -- L_35840165/LConn1
  T_35840165_380000_Leibstadt/RConn2 -- L_35840165/LConn2
  L_35840165/LConn3 -- T_35840165_380000_Leibstadt/RConn3 -- bus155/LConn1
  T_402055336__Gstaad/RConn1 -- L_402055336/LConn1
  T_402055336__Gstaad/RConn2 -- L_402055336/LConn2
  L_402055336/LConn3 -- T_402055336__Gstaad/RConn3 -- bus156/LConn1
  T_234983117__Chamoson/RConn1 -- L_234983117/LConn1
  T_234983117__Chamoson/RConn2 -- L_234983117/LConn2
  L_234983117/LConn3 -- T_234983117__Chamoson/RConn3 -- bus157/LConn1
  T_384104425__/RConn1 -- L_384104425/LConn1
  T_384104425__/RConn2 -- L_384104425/LConn2
  L_384104425/LConn3 -- T_384104425__/RConn3 -- bus158/LConn1
  T_165513396__/RConn1 -- L_165513396/LConn1
  T_165513396__/RConn2 -- L_165513396/LConn2
  L_165513396/LConn3 -- T_165513396__/RConn3 -- bus159/LConn1
  T_89405664_220000;132000;15000_Rupperswil/RConn1 -- L_89405664/LConn1
  T_89405664_220000;132000;15000_Rupperswil/RConn2 -- L_89405664/LConn2
  L_89405664/LConn3 -- T_89405664_220000;132000;15000_Rupperswil/RConn3 -- bus160/LConn1
  T_83861269_220000_Montlingen/RConn1 -- L_83861269/LConn1
  T_83861269_220000_Montlingen/RConn2 -- L_83861269/LConn2
  L_83861269/LConn3 -- T_83861269_220000_Montlingen/RConn3 -- bus161/LConn1
  T_92873516_220000_Mörschwil/RConn1 -- L_92873516/LConn1
  T_92873516_220000_Mörschwil/RConn2 -- L_92873516/LConn2
  L_92873516/LConn3 -- T_92873516_220000_Mörschwil/RConn3 -- bus162/LConn1
  T_212722603__/RConn1 -- L_212722603/LConn1
  T_212722603__/RConn2 -- L_212722603/LConn2
  L_212722603/LConn3 -- T_212722603__/RConn3 -- bus163/LConn1
  T_197031131__/RConn1 -- L_197031131/LConn1
  T_197031131__/RConn2 -- L_197031131/LConn2
  L_197031131/LConn3 -- T_197031131__/RConn3 -- bus164/LConn1
  T_190819048__Oftringen/RConn1 -- L_190819048/LConn1
  T_190819048__Oftringen/RConn2 -- L_190819048/LConn2
  L_190819048/LConn3 -- T_190819048__Oftringen/RConn3 -- bus165/LConn1
  T_207991759_380000_Robbia/RConn1 -- L_207991759/LConn1
  T_207991759_380000_Robbia/RConn2 -- L_207991759/LConn2
  L_207991759/LConn3 -- T_207991759_380000_Robbia/RConn3 -- bus166/LConn1
  T_402053379_220000_Lindenholz/RConn1 -- L_402053379/LConn1
  T_402053379_220000_Lindenholz/RConn2 -- L_402053379/LConn2
  L_402053379/LConn3 -- T_402053379_220000_Lindenholz/RConn3 -- bus167/LConn1
  T_164850030__Bickingen/RConn1 -- L_164850030/LConn1
  T_164850030__Bickingen/RConn2 -- L_164850030/LConn2
  L_164850030/LConn3 -- T_164850030__Bickingen/RConn3 -- bus168/LConn1
  T_236819191__/RConn1 -- L_236819191/LConn1
  T_236819191__/RConn2 -- L_236819191/LConn2
  L_236819191/LConn3 -- T_236819191__/RConn3 -- bus169/LConn1
  T_228003081__/RConn1 -- L_228003081/LConn1
  T_228003081__/RConn2 -- L_228003081/LConn2
  L_228003081/LConn3 -- T_228003081__/RConn3 -- bus170/LConn1
  T_109037817_220000_Lachmatt/RConn1 -- L_109037817/LConn1
  T_109037817_220000_Lachmatt/RConn2 -- L_109037817/LConn2
  L_109037817/LConn3 -- T_109037817_220000_Lachmatt/RConn3 -- bus171/LConn1
  T_109029720__Münchwilen/RConn1 -- L_109029720/LConn1
  T_109029720__Münchwilen/RConn2 -- L_109029720/LConn2
  L_109029720/LConn3 -- T_109029720__Münchwilen/RConn3 -- bus172/LConn1
  T_397960460_380000_Asphard/RConn1 -- L_397960460/LConn1
  T_397960460_380000_Asphard/RConn2 -- L_397960460/LConn2
  L_397960460/LConn3 -- T_397960460_380000_Asphard/RConn3 -- bus173/LConn1
  T_240959264__/RConn1 -- L_240959264/LConn1
  T_240959264__/RConn2 -- L_240959264/LConn2
  L_240959264/LConn3 -- T_240959264__/RConn3 -- bus174/LConn1
  T_26166640_220000_Unterstation_Wattenwil_(BKW_Energie)/RConn1 -- L_26166640/LConn1
  T_26166640_220000_Unterstation_Wattenwil_(BKW_Energie)/RConn2 -- L_26166640/LConn2
  L_26166640/LConn3 -- T_26166640_220000_Unterstation_Wattenwil_(BKW_Energie)/RConn3 -- bus175/LConn1
  T_161853746__/RConn1 -- L_161853746/LConn1
  T_161853746__/RConn2 -- L_161853746/LConn2
  L_161853746/LConn3 -- T_161853746__/RConn3 -- bus176/LConn1
  T_80266169__Mühleberg_West/RConn1 -- L_80266169/LConn1
  T_80266169__Mühleberg_West/RConn2 -- L_80266169/LConn2
  L_80266169/LConn3 -- T_80266169__Mühleberg_West/RConn3 -- bus177/LConn1
  T_100662075__Sedrun/RConn1 -- L_100662075/LConn1
  T_100662075__Sedrun/RConn2 -- L_100662075/LConn2
  L_100662075/LConn3 -- T_100662075__Sedrun/RConn3 -- bus178/LConn1
  T_27107779_220000_Eglisau/RConn1 -- L_27107779/LConn1
  T_27107779_220000_Eglisau/RConn2 -- L_27107779/LConn2
  L_27107779/LConn3 -- T_27107779_220000_Eglisau/RConn3 -- bus179/LConn1
  T_329659200__Lastverteilerwerk_Neubrück/RConn1 -- L_329659200/LConn1
  T_329659200__Lastverteilerwerk_Neubrück/RConn2 -- L_329659200/LConn2
  L_329659200/LConn3 -- T_329659200__Lastverteilerwerk_Neubrück/RConn3 -- bus180/LConn1
  T_34238394_220000_Mühleberg_Ost/RConn1 -- L_34238394/LConn1
  T_34238394_220000_Mühleberg_Ost/RConn2 -- L_34238394/LConn2
  L_34238394/LConn3 -- T_34238394_220000_Mühleberg_Ost/RConn3 -- bus181/LConn1
  T_87281514__/RConn1 -- L_87281514/LConn1
  T_87281514__/RConn2 -- L_87281514/LConn2
  L_87281514/LConn3 -- T_87281514__/RConn3 -- bus182/LConn1
  T_208623457__/RConn1 -- L_208623457/LConn1
  T_208623457__/RConn2 -- L_208623457/LConn2
  L_208623457/LConn3 -- T_208623457__/RConn3 -- bus183/LConn1
  T_196539748__/RConn1 -- L_196539748/LConn1
  T_196539748__/RConn2 -- L_196539748/LConn2
  L_196539748/LConn3 -- T_196539748__/RConn3 -- bus184/LConn1
  T_164850027__Bickigen/RConn1 -- L_164850027/LConn1
  T_164850027__Bickigen/RConn2 -- L_164850027/LConn2
  L_164850027/LConn3 -- T_164850027__Bickigen/RConn3 -- bus185/LConn1
  T_281804158__Soazza/RConn1 -- L_281804158/LConn1
  T_281804158__Soazza/RConn2 -- L_281804158/LConn2
  L_281804158/LConn3 -- T_281804158__Soazza/RConn3 -- bus186/LConn1
  T_35487135__/RConn1 -- L_35487135/LConn1
  T_35487135__/RConn2 -- L_35487135/LConn2
  L_35487135/LConn3 -- T_35487135__/RConn3 -- bus187/LConn1
  T_57038202__/RConn1 -- L_57038202/LConn1
  T_57038202__/RConn2 -- L_57038202/LConn2
  L_57038202/LConn3 -- T_57038202__/RConn3 -- bus188/LConn1
  T_57038204__/RConn1 -- L_57038204/LConn1
  T_57038204__/RConn2 -- L_57038204/LConn2
  L_57038204/LConn3 -- T_57038204__/RConn3 -- bus189/LConn1
  T_27435934_220000_Froloo/RConn1 -- L_27435934/LConn1
  T_27435934_220000_Froloo/RConn2 -- L_27435934/LConn2
  L_27435934/LConn3 -- T_27435934_220000_Froloo/RConn3 -- bus190/LConn1
  T_193131937__/RConn4 -- L_193131937/LConn1
  T_193131937__/RConn5 -- L_193131937/LConn2
  L_193131937/LConn3 -- T_193131937__/RConn6 -- bus191/LConn1
  T_163881972__/RConn1 -- L_163881972/LConn1
  T_163881972__/RConn2 -- L_163881972/LConn2
  L_163881972/LConn3 -- T_163881972__/RConn3 -- bus192/LConn1
